simulink model "Simulink_mg_1234_with_DistributedControl_ControlConmutado"  (R2018a)
settings: Solver=VariableStepAuto  StartTime=0.0  StopTime=50  FixedStep=1e-6  MaxStep=1e-3  RelTol=1e-3
values from neighbouring files (symbols this model uses):
  aij = 1    [Simulation_Base_4_mg.m]    (also in Simulation_alpha_vs_tau.m)
  aij_1 = 10    [Simulation_Base_4_mg.m]    (also in Simulation_alpha_vs_tau.m)
  aij_2 = 10    [Simulation_Base_4_mg.m]    (also in Simulation_alpha_vs_tau.m)
  aij_3 = 10    [Simulation_Base_4_mg.m]    (also in Simulation_alpha_vs_tau.m)
  aij_4 = 10    [Simulation_Base_4_mg.m]    (also in Simulation_alpha_vs_tau.m)
  C_mg_1 = Ctot .* dist    [Simulation_Base_4_mg.m]    (also in Simulation_alpha_vs_tau.m)
  C_mg_2 = Ctot .* dist    [Simulation_Base_4_mg.m]    (also in Simulation_alpha_vs_tau.m)
  C_mg_3 = Ctot .* dist    [Simulation_Base_4_mg.m]    (also in Simulation_alpha_vs_tau.m)
  C_mg_4 = Ctot .* dist    [Simulation_Base_4_mg.m]    (also in Simulation_alpha_vs_tau.m)
  g12 = 1.2    [Simulation_Base_4_mg.m]    (also in Simulation_alpha_vs_tau.m)
  g12_1 = 1/r_jk    (= 10)    [Simulation_Base_4_mg.m]    (also in Simulation_alpha_vs_tau.m)
  g12_2 = 1/r_jk    (= 10)    [Simulation_Base_4_mg.m]    (also in Simulation_alpha_vs_tau.m)
  g12_3 = 1/r_jk    (= 10)    [Simulation_Base_4_mg.m]    (also in Simulation_alpha_vs_tau.m)
  g12_4 = 1/r_jk    (= 10)    [Simulation_Base_4_mg.m]    (also in Simulation_alpha_vs_tau.m)
  g13 = ((0.383+1.756) / (0.383*1.756))^(-1)    (= 0.31442169238)    [Simulation_Base_4_mg.m]    (also in Simulation_alpha_vs_tau.m)
  g13_1 = 1/r_jk    (= 10)    [Simulation_Base_4_mg.m]    (also in Simulation_alpha_vs_tau.m)
  g13_3 = 1/r_jk    (= 10)    [Simulation_Base_4_mg.m]    (also in Simulation_alpha_vs_tau.m)
  g13_4 = 1/r_jk    (= 10)    [Simulation_Base_4_mg.m]    (also in Simulation_alpha_vs_tau.m)
  g23_1 = 1/r_jk    (= 10)    [Simulation_Base_4_mg.m]    (also in Simulation_alpha_vs_tau.m)
  g23_4 = 1/r_jk    (= 10)    [Simulation_Base_4_mg.m]    (also in Simulation_alpha_vs_tau.m)
  g24 = 1.55    [Simulation_Base_4_mg.m]    (also in Simulation_alpha_vs_tau.m)
  g24_3 = 1/r_jk    (= 10)    [Simulation_Base_4_mg.m]    (also in Simulation_alpha_vs_tau.m)
  g24_4 = 1/r_jk    (= 10)    [Simulation_Base_4_mg.m]    (also in Simulation_alpha_vs_tau.m)
  g34 = 0.75    [Simulation_Base_4_mg.m]    (also in Simulation_alpha_vs_tau.m)
  g34_3 = 1/r_jk    (= 10)    [Simulation_Base_4_mg.m]    (also in Simulation_alpha_vs_tau.m)
  g34_4 = 1/r_jk    (= 10)    [Simulation_Base_4_mg.m]    (also in Simulation_alpha_vs_tau.m)
  h = 0.99    [Simulation_Base_4_mg.m]    (also in Simulation_alpha_vs_tau.m)
  I_rate = [100,50,33,33]    [Simulation_Base_4_mg.m]    (also in Simulation_alpha_vs_tau.m)
  I_rate_1 = [5, 2.5, 2.5]    [Simulation_Base_4_mg.m]    (also in Simulation_alpha_vs_tau.m)
  I_rate_2 = [2.5, 5]    [Simulation_Base_4_mg.m]    (also in Simulation_alpha_vs_tau.m)
  I_rate_3 = [4, 3, 2, 1]    [Simulation_Base_4_mg.m]    (also in Simulation_alpha_vs_tau.m)
  I_rate_4 = [4, 3, 2, 1]    [Simulation_Base_4_mg.m]    (also in Simulation_alpha_vs_tau.m)
  k_ii = 60    [Simulation_Base_4_mg.m]    (also in Simulation_alpha_vs_tau.m)
  k_ii2 = 10    [Simulation_Base_4_mg.m]    (also in Simulation_alpha_vs_tau.m)
  k_ii_1 = 1000    [Simulation_Base_4_mg.m]    (also in Simulation_alpha_vs_tau.m)
  k_ii_2 = 1000    [Simulation_Base_4_mg.m]    (also in Simulation_alpha_vs_tau.m)
  k_ii_3 = 1000    [Simulation_Base_4_mg.m]    (also in Simulation_alpha_vs_tau.m)
  k_ii_4 = 1000    [Simulation_Base_4_mg.m]    (also in Simulation_alpha_vs_tau.m)
  k_iv = 3    [Simulation_Base_4_mg.m]    (also in Simulation_alpha_vs_tau.m = 1)
  k_iv_1 = 30    [Simulation_Base_4_mg.m]    (also in Simulation_alpha_vs_tau.m)
  k_iv_2 = 30    [Simulation_Base_4_mg.m]    (also in Simulation_alpha_vs_tau.m)
  k_iv_3 = 30    [Simulation_Base_4_mg.m]    (also in Simulation_alpha_vs_tau.m)
  k_iv_4 = 30    [Simulation_Base_4_mg.m]    (also in Simulation_alpha_vs_tau.m)
  k_pi = 30    [Simulation_Base_4_mg.m]    (also in Simulation_alpha_vs_tau.m = 25)
  k_pi2 = 0.5    [Simulation_Base_4_mg.m]    (also in Simulation_alpha_vs_tau.m)
  k_pi_1 = 10    [Simulation_Base_4_mg.m]    (also in Simulation_alpha_vs_tau.m)
  k_pi_2 = 10    [Simulation_Base_4_mg.m]    (also in Simulation_alpha_vs_tau.m)
  k_pi_3 = 10    [Simulation_Base_4_mg.m]    (also in Simulation_alpha_vs_tau.m)
  k_pi_4 = 10    [Simulation_Base_4_mg.m]    (also in Simulation_alpha_vs_tau.m)
  kd_1 = [5, 2.5, 2.5]    [Simulation_Base_4_mg.m]    (also in Simulation_alpha_vs_tau.m)
  kd_2 = [2.5, 50]    [Simulation_Base_4_mg.m]    (also in Simulation_alpha_vs_tau.m)
  kd_3 = [4, 3, 2, 1]    [Simulation_Base_4_mg.m]    (also in Simulation_alpha_vs_tau.m)
  kd_4 = [4, 3, 2, 1]    [Simulation_Base_4_mg.m]    (also in Simulation_alpha_vs_tau.m)
  L_mg_1 = ones(n) .* n .* Ltot    [Simulation_Base_4_mg.m]    (also in Simulation_alpha_vs_tau.m)
  L_mg_2 = ones(n) .* n .* Ltot    [Simulation_Base_4_mg.m]    (also in Simulation_alpha_vs_tau.m)
  L_mg_3 = ones(n) .* n .* Ltot    [Simulation_Base_4_mg.m]    (also in Simulation_alpha_vs_tau.m)
  L_mg_4 = ones(n) .* n .* Ltot    [Simulation_Base_4_mg.m]    (also in Simulation_alpha_vs_tau.m)
  P_load_vertex_1 = [   P_load_vertex_1;                                                 P_aux(i1,1) , P_aux(i2,2) , P_aux(i3,3) ]    [Simulation_Base_4_mg.m]    (also in Simulation_alpha_vs_tau.m)
  P_load_vertex_2 = [   P_load_vertex_2;                                                 P_aux(i1,1) , P_aux(i2,2) ]    [Simulation_Base_4_mg.m]    (also in Simulation_alpha_vs_tau.m)
  P_load_vertex_3 = [   P_load_vertex_3;                                                 P_aux(i1,1) , P_aux(i2,2) , P_aux(i3,3), P_aux(i4,4) ]    [Simulation_Base_4_mg.m]    (also in Simulation_alpha_vs_tau.m)
  P_load_vertex_4 = [   P_load_vertex_4;                                                 P_aux(i1,1) , P_aux(i2,2) , P_aux(i3,3), P_aux(i4,4) ]    [Simulation_Base_4_mg.m]    (also in Simulation_alpha_vs_tau.m)
  r_d0 = 1.3    [Simulation_Base_4_mg.m]    (also in Simulation_alpha_vs_tau.m)
  rd_mg_1 = n^2 * rtot .* dist    [Simulation_Base_4_mg.m]    (also in Simulation_alpha_vs_tau.m)
  rd_mg_2 = n^2 * rtot .* dist    [Simulation_Base_4_mg.m]    (also in Simulation_alpha_vs_tau.m)
  rd_mg_3 = n^2 * rtot .* dist    [Simulation_Base_4_mg.m]    (also in Simulation_alpha_vs_tau.m)
  rd_mg_4 = n^2 * rtot .* dist    [Simulation_Base_4_mg.m]    (also in Simulation_alpha_vs_tau.m)
  tau = 0.5    [Simulation_Base_4_mg.m]    (also in Simulation_alpha_vs_tau.m = 0.066)
  time_1 = 0.5    [Simulation_Base_4_mg.m]    (also in Simulation_alpha_vs_tau.m)
  time_2 = 15    [Simulation_Base_4_mg.m]    (also in Simulation_alpha_vs_tau.m = 5)
  time_4 = 5    [Simulation_Base_4_mg.m]    (also in Simulation_alpha_vs_tau.m = 15)
  time_6 = 50    [Simulation_Base_4_mg.m]    (also in Simulation_alpha_vs_tau.m = 13)
  time_7 = 50    [Simulation_Base_4_mg.m]    (also in Simulation_alpha_vs_tau.m = 100)
  time_8 = 50    [Simulation_Base_4_mg.m]    (also in Simulation_alpha_vs_tau.m = 100)
  time_9 = 100    [Simulation_Base_4_mg.m]    (also in Simulation_alpha_vs_tau.m)
  time_a_down = 100    [Simulation_alpha_vs_tau.m]
  time_a_up = 100    [Simulation_alpha_vs_tau.m]
  time_tau_down = 25    [Simulation_alpha_vs_tau.m]
  V_ref = 1050    [Simulation_Base_4_mg.m]    (also in Simulation_alpha_vs_tau.m)
undefined symbols (not defined in the file or in its folder): Zout_den_source, Zout_num_source
libraries: fl_lib x128, nesl_utility x89, elec_lib x26
(part 1 of 2)
settings Model: Creator=carna  LastModifiedBy=carna
settings SolverCC: ZeroCrossAlgorithm=Adaptive

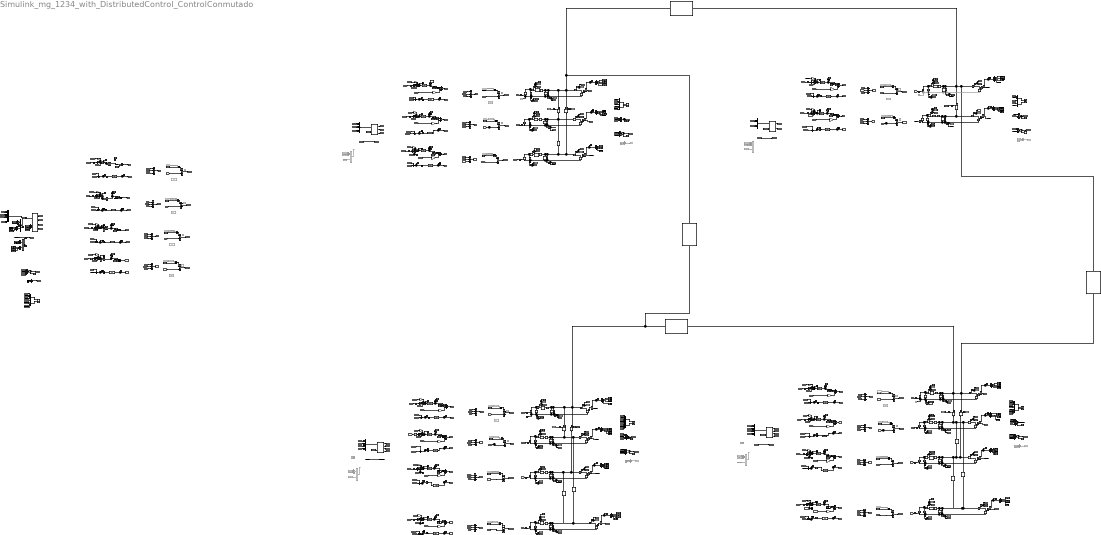
== system Simulink_mg_1234_with_DistributedControl_ControlConmutado ==
  note: Delta v 1
  note: Delta v 2
  note: DELTA I
  note: Delta R droop
  note: DELTA I
  note: Delta R droop
  note: Delta R droop
  note: DELTA I
  note: V MG
  note: I MG
  note: DELTA I
  note: Delta v 3
  note: Delta R droop
  note: Delta v 1
  note: Delta v 2
  note: DELTA I
  note: Delta R droop
  note: DELTA I
  note: Delta R droop
  note: Delta R droop
  note: DELTA I
  note: V MG
  note: I MG
  note: DELTA I
  note: Delta v 3
  note: Delta R droop
  note: Delta v 1
  note: Delta v 2
  note: DELTA I
  note: Delta R droop
  note: DELTA I
  note: Delta R droop
  note: Delta R droop
  note: DELTA I
  note: V MG
  note: I MG
  note: Delta v 1
  note: Delta v 2
  note: Delta R droop
  note: DELTA I
  note: Delta R droop
  note: DELTA I
  note: V MG
  note: I MG
  note: Delta v 1
  note: Delta R droop
  note: DELTA I
  note: V MG
  note: Delta v 1
  note: Delta R droop
  note: DELTA I
  note: Delta v 1
  note: Delta R droop
  note: DELTA I
  note: Delta v 1
  note: Delta R droop
  note: DELTA I
  Add{1,8,24,32,46..47,54,69} (8 alike) : Sum  Commented=on
  Add{2..4,9..13,15..16,19..20,36..38,61..62,73} (18 alike) : Sum  Inputs=++++
  Add{5,14,17,25..26,31,33,40..41,49,55,60,64..65,70,76,78} (17 alike) : Sum  Inputs=-+
  Add{6,18,22,27,29,39,43..44,50,52,57,63,67,71,75,77,79} (17 alike) : Sum  Inputs=-++
  Add{7,21,23,28,30,42,45,48,51,53,56,58..59,66,68,72,74,80} (18 alike) : Sum
  Add{34..35,81..83} (5 alike) : Sum  Inputs=+++
  C bus 1 : elec_lib/Passive Devices/Capacitor  enable_table=0  c=C_mg_3(1) F  Cvec=[1.0e-5, 1.0e-6] F  Vvec=[0.0, 10.0] V  CV_table_symmetry=1  C_tol=5  enable_C_tol=0  tol_distribution=1  nSigma=4  r=1e-6 Ohm  g=0 1/Ohm  enable_operating_limits=0  operating_limit_action=2  max_working_voltage_range=[-25.0, 25.0] V  power_rating=1 W  enable_faults=0  fault_action=1  Cscale_faulted=100  R_faulted=1e-3 Ohm  G_faulted=0 1/Ohm  tau_fault=1e-3 s  enable_temporal_fault=0  t_fault=1 s  enable_behavioral_fault=0  max_permissible_voltage_range=[-100.0, 100.0] V  t_fail_on_voltage=1 s  i_specify=off  i_priority=None  i=0 A  i_nominal_specify=off  i_nominal_unit=A  i_nominal_value=1  v_specify=off  v_priority=None  v=0 V  v_nominal_specify=off  v_nominal_unit=V  v_nominal_value=1  vc_specify=off  vc_priority=High  vc=0 V  vc_nominal_specify=off  vc_nominal_unit=V  vc_nominal_value=1
  C bus 10 : elec_lib/Passive Devices/Capacitor  enable_table=0  c=C_mg_1(2) F  Cvec=[1.0e-5, 1.0e-6] F  Vvec=[0.0, 10.0] V  CV_table_symmetry=1  C_tol=5  enable_C_tol=0  tol_distribution=1  nSigma=4  r=1e-6 Ohm  g=0 1/Ohm  enable_operating_limits=0  operating_limit_action=2  max_working_voltage_range=[-25.0, 25.0] V  power_rating=1 W  enable_faults=0  fault_action=1  Cscale_faulted=100  R_faulted=1e-3 Ohm  G_faulted=0 1/Ohm  tau_fault=1e-3 s  enable_temporal_fault=0  t_fault=1 s  enable_behavioral_fault=0  max_permissible_voltage_range=[-100.0, 100.0] V  t_fail_on_voltage=1 s  i_specify=off  i_priority=None  i=0 A  i_nominal_specify=off  i_nominal_unit=A  i_nominal_value=1  v_specify=on  v_priority=None  v=990 V  v_nominal_specify=off  v_nominal_unit=V  v_nominal_value=1  vc_specify=off  vc_priority=High  vc=0 V  vc_nominal_specify=off  vc_nominal_unit=V  vc_nominal_value=1
  C bus 11 : elec_lib/Passive Devices/Capacitor  enable_table=0  c=C_mg_1(3) F  Cvec=[1.0e-5, 1.0e-6] F  Vvec=[0.0, 10.0] V  CV_table_symmetry=1  C_tol=5  enable_C_tol=0  tol_distribution=1  nSigma=4  r=1e-6 Ohm  g=0 1/Ohm  enable_operating_limits=0  operating_limit_action=2  max_working_voltage_range=[-25.0, 25.0] V  power_rating=1 W  enable_faults=0  fault_action=1  Cscale_faulted=100  R_faulted=1e-3 Ohm  G_faulted=0 1/Ohm  tau_fault=1e-3 s  enable_temporal_fault=0  t_fault=1 s  enable_behavioral_fault=0  max_permissible_voltage_range=[-100.0, 100.0] V  t_fail_on_voltage=1 s  i_specify=off  i_priority=None  i=0 A  i_nominal_specify=off  i_nominal_unit=A  i_nominal_value=1  v_specify=on  v_priority=None  v=990 V  v_nominal_specify=off  v_nominal_unit=V  v_nominal_value=1  vc_specify=off  vc_priority=High  vc=0 V  vc_nominal_specify=off  vc_nominal_unit=V  vc_nominal_value=1
  C bus 12 : elec_lib/Passive Devices/Capacitor  enable_table=0  c=C_mg_2(2) F  Cvec=[1.0e-5, 1.0e-6] F  Vvec=[0.0, 10.0] V  CV_table_symmetry=1  C_tol=5  enable_C_tol=0  tol_distribution=1  nSigma=4  r=1e-6 Ohm  g=0 1/Ohm  enable_operating_limits=0  operating_limit_action=2  max_working_voltage_range=[-25.0, 25.0] V  power_rating=1 W  enable_faults=0  fault_action=1  Cscale_faulted=100  R_faulted=1e-3 Ohm  G_faulted=0 1/Ohm  tau_fault=1e-3 s  enable_temporal_fault=0  t_fault=1 s  enable_behavioral_fault=0  max_permissible_voltage_range=[-100.0, 100.0] V  t_fail_on_voltage=1 s  i_specify=off  i_priority=None  i=0 A  i_nominal_specify=off  i_nominal_unit=A  i_nominal_value=1  v_specify=on  v_priority=None  v=990 V  v_nominal_specify=off  v_nominal_unit=V  v_nominal_value=1  vc_specify=off  vc_priority=High  vc=0 V  vc_nominal_specify=off  vc_nominal_unit=V  vc_nominal_value=1
  C bus 14 : elec_lib/Passive Devices/Capacitor  enable_table=0  c=C_mg_2(1) F  Cvec=[1.0e-5, 1.0e-6] F  Vvec=[0.0, 10.0] V  CV_table_symmetry=1  C_tol=5  enable_C_tol=0  tol_distribution=1  nSigma=4  r=1e-6 Ohm  g=0 1/Ohm  enable_operating_limits=0  operating_limit_action=2  max_working_voltage_range=[-25.0, 25.0] V  power_rating=1 W  enable_faults=0  fault_action=1  Cscale_faulted=100  R_faulted=1e-3 Ohm  G_faulted=0 1/Ohm  tau_fault=1e-3 s  enable_temporal_fault=0  t_fault=1 s  enable_behavioral_fault=0  max_permissible_voltage_range=[-100.0, 100.0] V  t_fail_on_voltage=1 s  i_specify=off  i_priority=None  i=0 A  i_nominal_specify=off  i_nominal_unit=A  i_nominal_value=1  v_specify=on  v_priority=None  v=990 V  v_nominal_specify=off  v_nominal_unit=V  v_nominal_value=1  vc_specify=off  vc_priority=High  vc=0 V  vc_nominal_specify=off  vc_nominal_unit=V  vc_nominal_value=1
  C bus 2 : elec_lib/Passive Devices/Capacitor  enable_table=0  c=C_mg_3(2) F  Cvec=[1.0e-5, 1.0e-6] F  Vvec=[0.0, 10.0] V  CV_table_symmetry=1  C_tol=5  enable_C_tol=0  tol_distribution=1  nSigma=4  r=1e-6 Ohm  g=0 1/Ohm  enable_operating_limits=0  operating_limit_action=2  max_working_voltage_range=[-25.0, 25.0] V  power_rating=1 W  enable_faults=0  fault_action=1  Cscale_faulted=100  R_faulted=1e-3 Ohm  G_faulted=0 1/Ohm  tau_fault=1e-3 s  enable_temporal_fault=0  t_fault=1 s  enable_behavioral_fault=0  max_permissible_voltage_range=[-100.0, 100.0] V  t_fail_on_voltage=1 s  i_specify=off  i_priority=None  i=0 A  i_nominal_specify=off  i_nominal_unit=A  i_nominal_value=1  v_specify=off  v_priority=None  v=0 V  v_nominal_specify=off  v_nominal_unit=V  v_nominal_value=1  vc_specify=off  vc_priority=High  vc=0 V  vc_nominal_specify=off  vc_nominal_unit=V  vc_nominal_value=1
  C bus 3 : elec_lib/Passive Devices/Capacitor  enable_table=0  c=C_mg_3(3) F  Cvec=[1.0e-5, 1.0e-6] F  Vvec=[0.0, 10.0] V  CV_table_symmetry=1  C_tol=5  enable_C_tol=0  tol_distribution=1  nSigma=4  r=1e-6 Ohm  g=0 1/Ohm  enable_operating_limits=0  operating_limit_action=2  max_working_voltage_range=[-25.0, 25.0] V  power_rating=1 W  enable_faults=0  fault_action=1  Cscale_faulted=100  R_faulted=1e-3 Ohm  G_faulted=0 1/Ohm  tau_fault=1e-3 s  enable_temporal_fault=0  t_fault=1 s  enable_behavioral_fault=0  max_permissible_voltage_range=[-100.0, 100.0] V  t_fail_on_voltage=1 s  i_specify=off  i_priority=None  i=0 A  i_nominal_specify=off  i_nominal_unit=A  i_nominal_value=1  v_specify=off  v_priority=None  v=0 V  v_nominal_specify=off  v_nominal_unit=V  v_nominal_value=1  vc_specify=off  vc_priority=High  vc=0 V  vc_nominal_specify=off  vc_nominal_unit=V  vc_nominal_value=1
  C bus 4 : elec_lib/Passive Devices/Capacitor  enable_table=0  c=C_mg_3(4) F  Cvec=[1.0e-5, 1.0e-6] F  Vvec=[0.0, 10.0] V  CV_table_symmetry=1  C_tol=5  enable_C_tol=0  tol_distribution=1  nSigma=4  r=1e-6 Ohm  g=0 1/Ohm  enable_operating_limits=0  operating_limit_action=2  max_working_voltage_range=[-25.0, 25.0] V  power_rating=1 W  enable_faults=0  fault_action=1  Cscale_faulted=100  R_faulted=1e-3 Ohm  G_faulted=0 1/Ohm  tau_fault=1e-3 s  enable_temporal_fault=0  t_fault=1 s  enable_behavioral_fault=0  max_permissible_voltage_range=[-100.0, 100.0] V  t_fail_on_voltage=1 s  i_specify=off  i_priority=None  i=0 A  i_nominal_specify=off  i_nominal_unit=A  i_nominal_value=1  v_specify=off  v_priority=None  v=0 V  v_nominal_specify=off  v_nominal_unit=V  v_nominal_value=1  vc_specify=off  vc_priority=High  vc=0 V  vc_nominal_specify=off  vc_nominal_unit=V  vc_nominal_value=1
  C bus 5 : elec_lib/Passive Devices/Capacitor  enable_table=0  c=C_mg_3(1) F  Cvec=[1.0e-5, 1.0e-6] F  Vvec=[0.0, 10.0] V  CV_table_symmetry=1  C_tol=5  enable_C_tol=0  tol_distribution=1  nSigma=4  r=1e-6 Ohm  g=0 1/Ohm  enable_operating_limits=0  operating_limit_action=2  max_working_voltage_range=[-25.0, 25.0] V  power_rating=1 W  enable_faults=0  fault_action=1  Cscale_faulted=100  R_faulted=1e-3 Ohm  G_faulted=0 1/Ohm  tau_fault=1e-3 s  enable_temporal_fault=0  t_fault=1 s  enable_behavioral_fault=0  max_permissible_voltage_range=[-100.0, 100.0] V  t_fail_on_voltage=1 s  i_specify=off  i_priority=None  i=0 A  i_nominal_specify=off  i_nominal_unit=A  i_nominal_value=1  v_specify=off  v_priority=None  v=0 V  v_nominal_specify=off  v_nominal_unit=V  v_nominal_value=1  vc_specify=off  vc_priority=High  vc=0 V  vc_nominal_specify=off  vc_nominal_unit=V  vc_nominal_value=1
  C bus 6 : elec_lib/Passive Devices/Capacitor  enable_table=0  c=C_mg_4(2) F  Cvec=[1.0e-5, 1.0e-6] F  Vvec=[0.0, 10.0] V  CV_table_symmetry=1  C_tol=5  enable_C_tol=0  tol_distribution=1  nSigma=4  r=1e-6 Ohm  g=0 1/Ohm  enable_operating_limits=0  operating_limit_action=2  max_working_voltage_range=[-25.0, 25.0] V  power_rating=1 W  enable_faults=0  fault_action=1  Cscale_faulted=100  R_faulted=1e-3 Ohm  G_faulted=0 1/Ohm  tau_fault=1e-3 s  enable_temporal_fault=0  t_fault=1 s  enable_behavioral_fault=0  max_permissible_voltage_range=[-100.0, 100.0] V  t_fail_on_voltage=1 s  i_specify=off  i_priority=None  i=0 A  i_nominal_specify=off  i_nominal_unit=A  i_nominal_value=1  v_specify=off  v_priority=None  v=0 V  v_nominal_specify=off  v_nominal_unit=V  v_nominal_value=1  vc_specify=off  vc_priority=High  vc=0 V  vc_nominal_specify=off  vc_nominal_unit=V  vc_nominal_value=1
  C bus 7 : elec_lib/Passive Devices/Capacitor  enable_table=0  c=C_mg_3(3) F  Cvec=[1.0e-5, 1.0e-6] F  Vvec=[0.0, 10.0] V  CV_table_symmetry=1  C_tol=5  enable_C_tol=0  tol_distribution=1  nSigma=4  r=1e-6 Ohm  g=0 1/Ohm  enable_operating_limits=0  operating_limit_action=2  max_working_voltage_range=[-25.0, 25.0] V  power_rating=1 W  enable_faults=0  fault_action=1  Cscale_faulted=100  R_faulted=1e-3 Ohm  G_faulted=0 1/Ohm  tau_fault=1e-3 s  enable_temporal_fault=0  t_fault=1 s  enable_behavioral_fault=0  max_permissible_voltage_range=[-100.0, 100.0] V  t_fail_on_voltage=1 s  i_specify=off  i_priority=None  i=0 A  i_nominal_specify=off  i_nominal_unit=A  i_nominal_value=1  v_specify=off  v_priority=None  v=0 V  v_nominal_specify=off  v_nominal_unit=V  v_nominal_value=1  vc_specify=off  vc_priority=High  vc=0 V  vc_nominal_specify=off  vc_nominal_unit=V  vc_nominal_value=1
  C bus 8 : elec_lib/Passive Devices/Capacitor  enable_table=0  c=C_mg_4(4) F  Cvec=[1.0e-5, 1.0e-6] F  Vvec=[0.0, 10.0] V  CV_table_symmetry=1  C_tol=5  enable_C_tol=0  tol_distribution=1  nSigma=4  r=1e-6 Ohm  g=0 1/Ohm  enable_operating_limits=0  operating_limit_action=2  max_working_voltage_range=[-25.0, 25.0] V  power_rating=1 W  enable_faults=0  fault_action=1  Cscale_faulted=100  R_faulted=1e-3 Ohm  G_faulted=0 1/Ohm  tau_fault=1e-3 s  enable_temporal_fault=0  t_fault=1 s  enable_behavioral_fault=0  max_permissible_voltage_range=[-100.0, 100.0] V  t_fail_on_voltage=1 s  i_specify=off  i_priority=None  i=0 A  i_nominal_specify=off  i_nominal_unit=A  i_nominal_value=1  v_specify=off  v_priority=None  v=0 V  v_nominal_specify=off  v_nominal_unit=V  v_nominal_value=1  vc_specify=off  vc_priority=High  vc=0 V  vc_nominal_specify=off  vc_nominal_unit=V  vc_nominal_value=1
  C bus 9 : elec_lib/Passive Devices/Capacitor  enable_table=0  c=C_mg_1(1) F  Cvec=[1.0e-5, 1.0e-6] F  Vvec=[0.0, 10.0] V  CV_table_symmetry=1  C_tol=5  enable_C_tol=0  tol_distribution=1  nSigma=4  r=1e-6 Ohm  g=0 1/Ohm  enable_operating_limits=0  operating_limit_action=2  max_working_voltage_range=[-25.0, 25.0] V  power_rating=1 W  enable_faults=0  fault_action=1  Cscale_faulted=100  R_faulted=1e-3 Ohm  G_faulted=0 1/Ohm  tau_fault=1e-3 s  enable_temporal_fault=0  t_fault=1 s  enable_behavioral_fault=0  max_permissible_voltage_range=[-100.0, 100.0] V  t_fail_on_voltage=1 s  i_specify=off  i_priority=None  i=0 A  i_nominal_specify=off  i_nominal_unit=A  i_nominal_value=1  v_specify=on  v_priority=None  v=990 V  v_nominal_specify=off  v_nominal_unit=V  v_nominal_value=1  vc_specify=off  vc_priority=High  vc=0 V  vc_nominal_specify=off  vc_nominal_unit=V  vc_nominal_value=1
  Close loop equivalent{1..4} (4 alike) : TransferFcn  Numerator=[0 k_iv_3 ]  Denominator=[1 0]
  Close loop equivalent{6,9..11,14,18,20..23,25,29..31,35,38,41} (17 alike) : TransferFcn  Commented=on  Numerator=Zout_num_source  Denominator=Zout_den_source
  Close loop equivalent{5,8,12..13} (4 alike) : TransferFcn  Numerator=[0 k_iv_4 ]  Denominator=[1 0]
  Close loop equivalent15 : TransferFcn  Numerator=[0 k_iv_1 ]  Denominator=[1 0]
  Close loop equivalent{7,16,19,26..27,34,37,40} (8 alike) : TransferFcn  Commented=on  Numerator=[1 ]  Denominator=[tau 1]
  Close loop equivalent17 : TransferFcn  Numerator=[0 k_iv_1 ]  Denominator=[1 0]
  Close loop equivalent24 : TransferFcn  Numerator=[0 k_iv_1 ]  Denominator=[1 0]
  Close loop equivalent28 : TransferFcn  Numerator=[0 k_iv_2 ]  Denominator=[1 0]
  Close loop equivalent32 : TransferFcn  Numerator=[0 k_iv_2 ]  Denominator=[1 0]
  Close loop equivalent{33,36,39,42} (4 alike) : TransferFcn  Numerator=[0 k_iv ]  Denominator=[1 0]
  Constant{1,6,23,27} (4 alike) : Constant  Commented=on  Value=tau/2
  Constant{2..3,7..16,19..22,24..26,28..31,34..38,44..49} (34 alike) : Constant  Value=0
  Constant{4,17,32,39} (4 alike) : Constant  Commented=on  Value=V_ref
  Constant18 : Constant  Value=aij_4
  Constant33 : Constant  Value=aij_1
  Constant40 : Constant  Value=aij_2
  Constant41 : Constant  Value=tau*3/4
  Constant42 : Constant  Value=aij
  Constant43 : Constant  Value=V_ref
  Constant5 : Constant  Value=aij_3
  Constant50 : Constant  Value=tau*3/4
  Controlled Current Source{1..13} (13 alike) : fl_lib/Electrical/Electrical Sources/Controlled Current Source
  Controlled Voltage Source{,1..12} (13 alike) : fl_lib/Electrical/Electrical Sources/Controlled Voltage Source
  Current cloop transfer- Transport Delay{1..12} (12 alike) : TransportDelay  Commented=on  DelayTime=0.1e-3
  Current load {1..12,14} (13 alike) : fl_lib/Electrical/Electrical Sensors/Current Sensor
  Current output {1..19,21} (20 alike) : fl_lib/Electrical/Electrical Sensors/Current Sensor
  Derivative : Derivative  Commented=on
  Derivative1 : Derivative  Commented=on
  Display{,1..41,43..47,49..53,55..57,59,61..63} (59 alike) : Display
  Divide{1..13} (13 alike) : Product  Inputs=*/
  Electrical Reference{,1..10,12..13} (13 alike) : fl_lib/Electrical/Electrical Elements/Electrical Reference
  From{47,104,144,172} (4 alike) : From  Commented=on  GotoTag=io_source_2
  From{54,113,151,161,182,247,256,265} (8 alike) : From  Commented=on  GotoTag=io_source_1
  From{18,56,77,116,153} (5 alike) : From  Commented=on  GotoTag=io_source_3
  Gain1 : Gain  Gain=1/I_rate_3(4)
  Gain10 : Gain  Gain=r_d0/kd_4(1)
  Gain11 : Gain  Gain=r_d0/kd_4(4)
  Gain12 : Gain  Gain=1/I_rate_3(2)
  Gain13 : Gain  Gain=1/I_rate_3(3)
  Gain14 : Gain  Gain=1/4
  Gain15 : Gain  Gain=r_d0/kd_3(2)
  Gain16 : Gain  Gain=r_d0/kd_3(3)
  Gain17 : Gain  Gain=1/I_rate_3(1)
  Gain18 : Gain  Gain=r_d0/kd_3(1)
  Gain19 : Gain  Gain=1/I_rate_2(2)
  Gain2 : Gain  Gain=r_d0/kd_3(4)
  Gain20 : Gain  Gain=1/I_rate_1(2)
  Gain21 : Gain  Gain=1/I_rate_1(3)
  Gain22 : Gain  Gain=r_d0/kd_1(2)
  Gain23 : Gain  Gain=r_d0/kd_1(3)
  Gain24 : Gain  Gain=1/I_rate_1(1)
  Gain25 : Gain  Gain=r_d0/kd_1(1)
  Gain26 : Gain  Gain=1/I_rate(1)
  Gain27 : Gain  Gain=1/3
  Gain28 : Gain  Gain=r_d0/kd_2(2)
  Gain29 : Gain  Gain=1/I_rate(2)
  Gain3 : Gain  Gain=1/I_rate_4(4)
  Gain30 : Gain  Gain=1/I_rate_2(1)
  Gain31 : Gain  Gain=r_d0/kd_2(1)
  Gain32 : Gain  Gain=1/2
  Gain33 : Gain  Gain=1/4
  Gain34 : Gain  Gain=1/I_rate(3)
  Gain35 : Gain  Gain=1/I_rate(4)
  Gain4 : Gain  Gain=1/I_rate_4(2)
  Gain5 : Gain  Gain=1/4
  Gain6 : Gain  Gain=1/I_rate_4(3)
  Gain7 : Gain  Gain=r_d0/kd_4(2)
  Gain8 : Gain  Gain=r_d0/kd_4(3)
  Gain9 : Gain  Gain=1/I_rate_4(1)
  Goto{29,44,94,106} (4 alike) : Goto  Commented=on  GotoTag=V_REF_c
  Integrator{1..17} (17 alike) : Integrator
  L serie 1 : elec_lib/Passive Devices/Inductor  l=L_mg_3(1) H  L_tol=20  enable_L_tol=0  tol_distribution=1  nSigma=4  r=0 Ohm  g=1e-9 1/Ohm  enable_operating_limits=0  operating_limit_action=2  max_working_current=1 A  power_rating=1 W  enable_faults=0  fault_action=1  lambdaPercent=50  k_faulted=0.9999  turnsShort=0  openCct=0  groundShort=0  groundShortG=0 1/Ohm  tau_fault=1e-3 s  enable_temporal_fault=0  t_fault=1 s  enable_behavioral_fault=0  max_permissible_voltage=100 V  n_fail_on_voltage=1  max_permissible_current=1 A  t_fail_on_current=1 s  i_L_specify=off  i_L_priority=High  i_L=0 A  i_L_nominal_specify=off  i_L_nominal_unit=A  i_L_nominal_value=1
      settings: SourceProductName=Simscape Electronics  SourceProductBaseCode=SN
  L serie 10 : elec_lib/Passive Devices/Inductor  l=L_mg_1(2) H  L_tol=20  enable_L_tol=0  tol_distribution=1  nSigma=4  r=0 Ohm  g=1e-9 1/Ohm  enable_operating_limits=0  operating_limit_action=2  max_working_current=1 A  power_rating=1 W  enable_faults=0  fault_action=1  lambdaPercent=50  k_faulted=0.9999  turnsShort=0  openCct=0  groundShort=0  groundShortG=0 1/Ohm  tau_fault=1e-3 s  enable_temporal_fault=0  t_fault=1 s  enable_behavioral_fault=0  max_permissible_voltage=100 V  n_fail_on_voltage=1  max_permissible_current=1 A  t_fail_on_current=1 s  i_L_specify=off  i_L_priority=High  i_L=0 A  i_L_nominal_specify=off  i_L_nominal_unit=A  i_L_nominal_value=1
      settings: SourceProductName=Simscape Electronics  SourceProductBaseCode=SN
  L serie 11 : elec_lib/Passive Devices/Inductor  l=L_mg_1(3) H  L_tol=20  enable_L_tol=0  tol_distribution=1  nSigma=4  r=0 Ohm  g=1e-9 1/Ohm  enable_operating_limits=0  operating_limit_action=2  max_working_current=1 A  power_rating=1 W  enable_faults=0  fault_action=1  lambdaPercent=50  k_faulted=0.9999  turnsShort=0  openCct=0  groundShort=0  groundShortG=0 1/Ohm  tau_fault=1e-3 s  enable_temporal_fault=0  t_fault=1 s  enable_behavioral_fault=0  max_permissible_voltage=100 V  n_fail_on_voltage=1  max_permissible_current=1 A  t_fail_on_current=1 s  i_L_specify=off  i_L_priority=High  i_L=0 A  i_L_nominal_specify=off  i_L_nominal_unit=A  i_L_nominal_value=1
      settings: SourceProductName=Simscape Electronics  SourceProductBaseCode=SN
  L serie 12 : elec_lib/Passive Devices/Inductor  l=L_mg_2(2) H  L_tol=20  enable_L_tol=0  tol_distribution=1  nSigma=4  r=0 Ohm  g=1e-9 1/Ohm  enable_operating_limits=0  operating_limit_action=2  max_working_current=1 A  power_rating=1 W  enable_faults=0  fault_action=1  lambdaPercent=50  k_faulted=0.9999  turnsShort=0  openCct=0  groundShort=0  groundShortG=0 1/Ohm  tau_fault=1e-3 s  enable_temporal_fault=0  t_fault=1 s  enable_behavioral_fault=0  max_permissible_voltage=100 V  n_fail_on_voltage=1  max_permissible_current=1 A  t_fail_on_current=1 s  i_L_specify=off  i_L_priority=High  i_L=0 A  i_L_nominal_specify=off  i_L_nominal_unit=A  i_L_nominal_value=1
      settings: SourceProductName=Simscape Electronics  SourceProductBaseCode=SN
  L serie 14 : elec_lib/Passive Devices/Inductor  l=L_mg_2(1) H  L_tol=20  enable_L_tol=0  tol_distribution=1  nSigma=4  r=0 Ohm  g=1e-9 1/Ohm  enable_operating_limits=0  operating_limit_action=2  max_working_current=1 A  power_rating=1 W  enable_faults=0  fault_action=1  lambdaPercent=50  k_faulted=0.9999  turnsShort=0  openCct=0  groundShort=0  groundShortG=0 1/Ohm  tau_fault=1e-3 s  enable_temporal_fault=0  t_fault=1 s  enable_behavioral_fault=0  max_permissible_voltage=100 V  n_fail_on_voltage=1  max_permissible_current=1 A  t_fail_on_current=1 s  i_L_specify=off  i_L_priority=High  i_L=0 A  i_L_nominal_specify=off  i_L_nominal_unit=A  i_L_nominal_value=1
      settings: SourceProductName=Simscape Electronics  SourceProductBaseCode=SN
  L serie 2 : elec_lib/Passive Devices/Inductor  l=L_mg_3(2) H  L_tol=20  enable_L_tol=0  tol_distribution=1  nSigma=4  r=0 Ohm  g=1e-9 1/Ohm  enable_operating_limits=0  operating_limit_action=2  max_working_current=1 A  power_rating=1 W  enable_faults=0  fault_action=1  lambdaPercent=50  k_faulted=0.9999  turnsShort=0  openCct=0  groundShort=0  groundShortG=0 1/Ohm  tau_fault=1e-3 s  enable_temporal_fault=0  t_fault=1 s  enable_behavioral_fault=0  max_permissible_voltage=100 V  n_fail_on_voltage=1  max_permissible_current=1 A  t_fail_on_current=1 s  i_L_specify=off  i_L_priority=High  i_L=0 A  i_L_nominal_specify=off  i_L_nominal_unit=A  i_L_nominal_value=1
      settings: SourceProductName=Simscape Electronics  SourceProductBaseCode=SN
  L serie 3 : elec_lib/Passive Devices/Inductor  l=L_mg_3(3) H  L_tol=20  enable_L_tol=0  tol_distribution=1  nSigma=4  r=0 Ohm  g=1e-9 1/Ohm  enable_operating_limits=0  operating_limit_action=2  max_working_current=1 A  power_rating=1 W  enable_faults=0  fault_action=1  lambdaPercent=50  k_faulted=0.9999  turnsShort=0  openCct=0  groundShort=0  groundShortG=0 1/Ohm  tau_fault=1e-3 s  enable_temporal_fault=0  t_fault=1 s  enable_behavioral_fault=0  max_permissible_voltage=100 V  n_fail_on_voltage=1  max_permissible_current=1 A  t_fail_on_current=1 s  i_L_specify=off  i_L_priority=High  i_L=0 A  i_L_nominal_specify=off  i_L_nominal_unit=A  i_L_nominal_value=1
      settings: SourceProductName=Simscape Electronics  SourceProductBaseCode=SN
  L serie 4 : elec_lib/Passive Devices/Inductor  l=L_mg_3(4) H  L_tol=20  enable_L_tol=0  tol_distribution=1  nSigma=4  r=0 Ohm  g=1e-9 1/Ohm  enable_operating_limits=0  operating_limit_action=2  max_working_current=1 A  power_rating=1 W  enable_faults=0  fault_action=1  lambdaPercent=50  k_faulted=0.9999  turnsShort=0  openCct=0  groundShort=0  groundShortG=0 1/Ohm  tau_fault=1e-3 s  enable_temporal_fault=0  t_fault=1 s  enable_behavioral_fault=0  max_permissible_voltage=100 V  n_fail_on_voltage=1  max_permissible_current=1 A  t_fail_on_current=1 s  i_L_specify=off  i_L_priority=High  i_L=0 A  i_L_nominal_specify=off  i_L_nominal_unit=A  i_L_nominal_value=1
      settings: SourceProductName=Simscape Electronics  SourceProductBaseCode=SN
  L serie 5 : elec_lib/Passive Devices/Inductor  l=L_mg_3(1) H  L_tol=20  enable_L_tol=0  tol_distribution=1  nSigma=4  r=0 Ohm  g=1e-9 1/Ohm  enable_operating_limits=0  operating_limit_action=2  max_working_current=1 A  power_rating=1 W  enable_faults=0  fault_action=1  lambdaPercent=50  k_faulted=0.9999  turnsShort=0  openCct=0  groundShort=0  groundShortG=0 1/Ohm  tau_fault=1e-3 s  enable_temporal_fault=0  t_fault=1 s  enable_behavioral_fault=0  max_permissible_voltage=100 V  n_fail_on_voltage=1  max_permissible_current=1 A  t_fail_on_current=1 s  i_L_specify=off  i_L_priority=High  i_L=0 A  i_L_nominal_specify=off  i_L_nominal_unit=A  i_L_nominal_value=1
      settings: SourceProductName=Simscape Electronics  SourceProductBaseCode=SN
  L serie 6 : elec_lib/Passive Devices/Inductor  l=L_mg_4(2) H  L_tol=20  enable_L_tol=0  tol_distribution=1  nSigma=4  r=0 Ohm  g=1e-9 1/Ohm  enable_operating_limits=0  operating_limit_action=2  max_working_current=1 A  power_rating=1 W  enable_faults=0  fault_action=1  lambdaPercent=50  k_faulted=0.9999  turnsShort=0  openCct=0  groundShort=0  groundShortG=0 1/Ohm  tau_fault=1e-3 s  enable_temporal_fault=0  t_fault=1 s  enable_behavioral_fault=0  max_permissible_voltage=100 V  n_fail_on_voltage=1  max_permissible_current=1 A  t_fail_on_current=1 s  i_L_specify=off  i_L_priority=High  i_L=0 A  i_L_nominal_specify=off  i_L_nominal_unit=A  i_L_nominal_value=1
      settings: SourceProductName=Simscape Electronics  SourceProductBaseCode=SN
  L serie 7 : elec_lib/Passive Devices/Inductor  l=L_mg_4(3) H  L_tol=20  enable_L_tol=0  tol_distribution=1  nSigma=4  r=0 Ohm  g=1e-9 1/Ohm  enable_operating_limits=0  operating_limit_action=2  max_working_current=1 A  power_rating=1 W  enable_faults=0  fault_action=1  lambdaPercent=50  k_faulted=0.9999  turnsShort=0  openCct=0  groundShort=0  groundShortG=0 1/Ohm  tau_fault=1e-3 s  enable_temporal_fault=0  t_fault=1 s  enable_behavioral_fault=0  max_permissible_voltage=100 V  n_fail_on_voltage=1  max_permissible_current=1 A  t_fail_on_current=1 s  i_L_specify=off  i_L_priority=High  i_L=0 A  i_L_nominal_specify=off  i_L_nominal_unit=A  i_L_nominal_value=1
      settings: SourceProductName=Simscape Electronics  SourceProductBaseCode=SN
  L serie 8 : elec_lib/Passive Devices/Inductor  l=L_mg_4(4) H  L_tol=20  enable_L_tol=0  tol_distribution=1  nSigma=4  r=0 Ohm  g=1e-9 1/Ohm  enable_operating_limits=0  operating_limit_action=2  max_working_current=1 A  power_rating=1 W  enable_faults=0  fault_action=1  lambdaPercent=50  k_faulted=0.9999  turnsShort=0  openCct=0  groundShort=0  groundShortG=0 1/Ohm  tau_fault=1e-3 s  enable_temporal_fault=0  t_fault=1 s  enable_behavioral_fault=0  max_permissible_voltage=100 V  n_fail_on_voltage=1  max_permissible_current=1 A  t_fail_on_current=1 s  i_L_specify=off  i_L_priority=High  i_L=0 A  i_L_nominal_specify=off  i_L_nominal_unit=A  i_L_nominal_value=1
      settings: SourceProductName=Simscape Electronics  SourceProductBaseCode=SN
  L serie 9 : elec_lib/Passive Devices/Inductor  l=L_mg_1(1) H  L_tol=20  enable_L_tol=0  tol_distribution=1  nSigma=4  r=0 Ohm  g=1e-9 1/Ohm  enable_operating_limits=0  operating_limit_action=2  max_working_current=1 A  power_rating=1 W  enable_faults=0  fault_action=1  lambdaPercent=50  k_faulted=0.9999  turnsShort=0  openCct=0  groundShort=0  groundShortG=0 1/Ohm  tau_fault=1e-3 s  enable_temporal_fault=0  t_fault=1 s  enable_behavioral_fault=0  max_permissible_voltage=100 V  n_fail_on_voltage=1  max_permissible_current=1 A  t_fail_on_current=1 s  i_L_specify=off  i_L_priority=High  i_L=0 A  i_L_nominal_specify=off  i_L_nominal_unit=A  i_L_nominal_value=1
      settings: SourceProductName=Simscape Electronics  SourceProductBaseCode=SN
  MATLAB Function1 : MATLAB Function  TreatAsAtomicUnit=on
  MATLAB Function2 : MATLAB Function  TreatAsAtomicUnit=on
  MATLAB Function3 : MATLAB Function  TreatAsAtomicUnit=on
  MATLAB Function4 : MATLAB Function  TreatAsAtomicUnit=on
  MATLAB Function5 : MATLAB Function  TreatAsAtomicUnit=on
  Manual Switch{1..17} (17 alike) : ManualSwitch  CurrentSetting=0
  Mux{,2,4,6..7,12..13} (7 alike) : Mux
  Mux1 : Mux  Inputs=5
  Mux10 : Mux  Inputs=3
  Mux11 : Mux  Inputs=2
  Mux14 : Mux  Inputs=5
  Mux3 : Mux  Inputs=5
  Mux5 : Mux  Inputs=3
  Mux8 : Mux  Inputs=3
  Mux9 : Mux  Inputs=2
  PI i 1 : TransferFcn  Numerator=[k_pi_4 k_ii_4 ]  Denominator=[1 0]
  PI i 2 : TransferFcn  Numerator=[k_pi_1 k_ii_1 ]  Denominator=[1 0]
  PI i 3 : TransferFcn  Numerator=[k_pi_3 k_ii_3 ]  Denominator=[1 0]
  PI i 4 : TransferFcn  Numerator=[k_pi_2 k_ii_2 ]  Denominator=[1 0]
  PI i1 : TransferFcn  Numerator=[k_pi_3 k_ii_3 ]  Denominator=[1 0]
  PI i2 : TransferFcn  Numerator=[k_pi_4 k_ii_4 ]  Denominator=[1 0]
  PI i3 : TransferFcn  Numerator=[k_pi_4 k_ii_4]  Denominator=[1 0]
  PI i4 : TransferFcn  Numerator=[k_pi_3 k_ii_3]  Denominator=[1 0]
  PI i5 : TransferFcn  Numerator=[k_pi_3 k_ii_3 ]  Denominator=[1 0]
  PI i6 : TransferFcn  Numerator=[k_pi_4 k_ii_4 ]  Denominator=[1 0]
  PI i7 : TransferFcn  Numerator=[k_pi_2 k_ii_2]  Denominator=[1 0]
  PI i8 : TransferFcn  Numerator=[k_pi_1 k_ii_1]  Denominator=[1 0]
  PI i9 : TransferFcn  Numerator=[k_pi_1 k_ii_1 ]  Denominator=[1 0]
  PS-Simulink Converter{,1..55,60..62} (59 alike) : nesl_utility/PS-Simulink Converter  PhysicalDomain=network_engine_domain  SubClassName=ps_output  LeftPortType=input  RightPortType=output  PseudoPeriodic=off  Frequencies=[]  Unit=1  AffineConversion=off
  Product{1..4} (4 alike) : Product  Commented=on
  Product5 : Product
  Product6 : Product
  R serie 1 : fl_lib/Electrical/Electrical Elements/Resistor  R=rd_mg_3(1) Ohm  i_specify=off  i_priority=None  i=0 A  i_nominal_specify=off  i_nominal_unit=A  i_nominal_value=1  v_specify=off  v_priority=None  v=0 V  v_nominal_specify=off  v_nominal_unit=V  v_nominal_value=1
  R serie 10 : fl_lib/Electrical/Electrical Elements/Resistor  R=rd_mg_4(2) Ohm  i_specify=off  i_priority=None  i=0 A  i_nominal_specify=off  i_nominal_unit=A  i_nominal_value=1  v_specify=off  v_priority=None  v=0 V  v_nominal_specify=off  v_nominal_unit=V  v_nominal_value=1
  R serie 11 : fl_lib/Electrical/Electrical Elements/Resistor  R=rd_mg_4(3) Ohm  i_specify=off  i_priority=None  i=0 A  i_nominal_specify=off  i_nominal_unit=A  i_nominal_value=1  v_specify=off  v_priority=None  v=0 V  v_nominal_specify=off  v_nominal_unit=V  v_nominal_value=1
  R serie 12 : fl_lib/Electrical/Electrical Elements/Resistor  R=1/(g12_3) Ohm  i_specify=off  i_priority=None  i=0 A  i_nominal_specify=off  i_nominal_unit=A  i_nominal_value=1  v_specify=off  v_priority=None  v=0 V  v_nominal_specify=off  v_nominal_unit=V  v_nominal_value=1
  R serie 13 : fl_lib/Electrical/Electrical Elements/Resistor  R=1/(g13_3) Ohm  i_specify=off  i_priority=None  i=0 A  i_nominal_specify=off  i_nominal_unit=A  i_nominal_value=1  v_specify=off  v_priority=None  v=0 V  v_nominal_specify=off  v_nominal_unit=V  v_nominal_value=1
  R serie 14 : fl_lib/Electrical/Electrical Elements/Resistor  R=rd_mg_4(4) Ohm  i_specify=off  i_priority=None  i=0 A  i_nominal_specify=off  i_nominal_unit=A  i_nominal_value=1  v_specify=off  v_priority=None  v=0 V  v_nominal_specify=off  v_nominal_unit=V  v_nominal_value=1
  R serie 15 : fl_lib/Electrical/Electrical Elements/Resistor  R=1/(g24_4) Ohm  i_specify=off  i_priority=None  i=0 A  i_nominal_specify=off  i_nominal_unit=A  i_nominal_value=1  v_specify=off  v_priority=None  v=0 V  v_nominal_specify=off  v_nominal_unit=V  v_nominal_value=1
  R serie 16 : fl_lib/Electrical/Electrical Elements/Resistor  R=1/(g34_4) Ohm  i_specify=off  i_priority=None  i=0 A  i_nominal_specify=off  i_nominal_unit=A  i_nominal_value=1  v_specify=off  v_priority=None  v=0 V  v_nominal_specify=off  v_nominal_unit=V  v_nominal_value=1
  R serie 17 : fl_lib/Electrical/Electrical Elements/Resistor  R=1/(g23_4) Ohm  i_specify=off  i_priority=None  i=0 A  i_nominal_specify=off  i_nominal_unit=A  i_nominal_value=1  v_specify=off  v_priority=None  v=0 V  v_nominal_specify=off  v_nominal_unit=V  v_nominal_value=1
  R serie 18 : fl_lib/Electrical/Electrical Elements/Resistor  R=1/g34 Ohm  i_specify=off  i_priority=None  i=0 A  i_nominal_specify=off  i_nominal_unit=A  i_nominal_value=1  v_specify=off  v_priority=None  v=0 V  v_nominal_specify=off  v_nominal_unit=V  v_nominal_value=1
  R serie 19 : fl_lib/Electrical/Electrical Elements/Resistor  R=rd_mg_1(1) Ohm  i_specify=off  i_priority=None  i=0 A  i_nominal_specify=off  i_nominal_unit=A  i_nominal_value=1  v_specify=off  v_priority=None  v=0 V  v_nominal_specify=off  v_nominal_unit=V  v_nominal_value=1
  R serie 2 : fl_lib/Electrical/Electrical Elements/Resistor  R=rd_mg_3(2) Ohm  i_specify=off  i_priority=None  i=0 A  i_nominal_specify=off  i_nominal_unit=A  i_nominal_value=1  v_specify=off  v_priority=None  v=0 V  v_nominal_specify=off  v_nominal_unit=V  v_nominal_value=1
  R serie 20 : fl_lib/Electrical/Electrical Elements/Resistor  R=1/(g12_1) Ohm  i_specify=off  i_priority=None  i=0 A  i_nominal_specify=off  i_nominal_unit=A  i_nominal_value=1  v_specify=off  v_priority=None  v=0 V  v_nominal_specify=off  v_nominal_unit=V  v_nominal_value=1
  R serie 21 : fl_lib/Electrical/Electrical Elements/Resistor  R=1/(g13_1) Ohm  i_specify=off  i_priority=None  i=0 A  i_nominal_specify=off  i_nominal_unit=A  i_nominal_value=1  v_specify=off  v_priority=None  v=0 V  v_nominal_specify=off  v_nominal_unit=V  v_nominal_value=1
  R serie 22 : fl_lib/Electrical/Electrical Elements/Resistor  R=rd_mg_1(2) Ohm  i_specify=off  i_priority=None  i=0 A  i_nominal_specify=off  i_nominal_unit=A  i_nominal_value=1  v_specify=off  v_priority=None  v=0 V  v_nominal_specify=off  v_nominal_unit=V  v_nominal_value=1
  R serie 23 : fl_lib/Electrical/Electrical Elements/Resistor  R=rd_mg_1(3) Ohm  i_specify=off  i_priority=None  i=0 A  i_nominal_specify=off  i_nominal_unit=A  i_nominal_value=1  v_specify=off  v_priority=None  v=0 V  v_nominal_specify=off  v_nominal_unit=V  v_nominal_value=1
  R serie 24 : fl_lib/Electrical/Electrical Elements/Resistor  R=rd_mg_2(1) Ohm  i_specify=off  i_priority=None  i=0 A  i_nominal_specify=off  i_nominal_unit=A  i_nominal_value=1  v_specify=off  v_priority=None  v=0 V  v_nominal_specify=off  v_nominal_unit=V  v_nominal_value=1
  R serie 25 : fl_lib/Electrical/Electrical Elements/Resistor  R=1/(g12_2) Ohm  i_specify=off  i_priority=None  i=0 A  i_nominal_specify=off  i_nominal_unit=A  i_nominal_value=1  v_specify=off  v_priority=None  v=0 V  v_nominal_specify=off  v_nominal_unit=V  v_nominal_value=1
  R serie 26 : fl_lib/Electrical/Electrical Elements/Resistor  R=1/(g23_1) Ohm  i_specify=off  i_priority=None  i=0 A  i_nominal_specify=off  i_nominal_unit=A  i_nominal_value=1  v_specify=off  v_priority=None  v=0 V  v_nominal_specify=off  v_nominal_unit=V  v_nominal_value=1
  R serie 27 : fl_lib/Electrical/Electrical Elements/Resistor  R=1/g12 Ohm  i_specify=off  i_priority=None  i=0 A  i_nominal_specify=off  i_nominal_unit=A  i_nominal_value=1  v_specify=off  v_priority=None  v=0 V  v_nominal_specify=off  v_nominal_unit=V  v_nominal_value=1
  R serie 28 : fl_lib/Electrical/Electrical Elements/Resistor  R=rd_mg_2(2) Ohm  i_specify=off  i_priority=None  i=0 A  i_nominal_specify=off  i_nominal_unit=A  i_nominal_value=1  v_specify=off  v_priority=None  v=0 V  v_nominal_specify=off  v_nominal_unit=V  v_nominal_value=1
  R serie 29 : fl_lib/Electrical/Electrical Elements/Resistor  R=1/g24 Ohm  i_specify=off  i_priority=None  i=0 A  i_nominal_specify=off  i_nominal_unit=A  i_nominal_value=1  v_specify=off  v_priority=None  v=0 V  v_nominal_specify=off  v_nominal_unit=V  v_nominal_value=1
  R serie 3 : fl_lib/Electrical/Electrical Elements/Resistor  R=rd_mg_3(3) Ohm  i_specify=off  i_priority=None  i=0 A  i_nominal_specify=off  i_nominal_unit=A  i_nominal_value=1  v_specify=off  v_priority=None  v=0 V  v_nominal_specify=off  v_nominal_unit=V  v_nominal_value=1
  R serie 30 : fl_lib/Electrical/Electrical Elements/Resistor  R=1/g13 Ohm  i_specify=off  i_priority=None  i=0 A  i_nominal_specify=off  i_nominal_unit=A  i_nominal_value=1  v_specify=off  v_priority=None  v=0 V  v_nominal_specify=off  v_nominal_unit=V  v_nominal_value=1
  R serie 4 : fl_lib/Electrical/Electrical Elements/Resistor  R=rd_mg_3(4) Ohm  i_specify=off  i_priority=None  i=0 A  i_nominal_specify=off  i_nominal_unit=A  i_nominal_value=1  v_specify=off  v_priority=None  v=0 V  v_nominal_specify=off  v_nominal_unit=V  v_nominal_value=1
  R serie 5 : fl_lib/Electrical/Electrical Elements/Resistor  R=1/(g24_3) Ohm  i_specify=off  i_priority=None  i=0 A  i_nominal_specify=off  i_nominal_unit=A  i_nominal_value=1  v_specify=off  v_priority=None  v=0 V  v_nominal_specify=off  v_nominal_unit=V  v_nominal_value=1
  R serie 6 : fl_lib/Electrical/Electrical Elements/Resistor  R=1/(g34_3) Ohm  i_specify=off  i_priority=None  i=0 A  i_nominal_specify=off  i_nominal_unit=A  i_nominal_value=1  v_specify=off  v_priority=None  v=0 V  v_nominal_specify=off  v_nominal_unit=V  v_nominal_value=1
  R serie 7 : fl_lib/Electrical/Electrical Elements/Resistor  R=rd_mg_3(1) Ohm  i_specify=off  i_priority=None  i=0 A  i_nominal_specify=off  i_nominal_unit=A  i_nominal_value=1  v_specify=off  v_priority=None  v=0 V  v_nominal_specify=off  v_nominal_unit=V  v_nominal_value=1
  R serie 8 : fl_lib/Electrical/Electrical Elements/Resistor  R=1/(g12_4) Ohm  i_specify=off  i_priority=None  i=0 A  i_nominal_specify=off  i_nominal_unit=A  i_nominal_value=1  v_specify=off  v_priority=None  v=0 V  v_nominal_specify=off  v_nominal_unit=V  v_nominal_value=1
  R serie 9 : fl_lib/Electrical/Electrical Elements/Resistor  R=1/(g13_4) Ohm  i_specify=off  i_priority=None  i=0 A  i_nominal_specify=off  i_nominal_unit=A  i_nominal_value=1  v_specify=off  v_priority=None  v=0 V  v_nominal_specify=off  v_nominal_unit=V  v_nominal_value=1
  Saturation{1..51} (51 alike) : Saturate  UpperLimit=100  LowerLimit=-100
  Scope{,9,48..49,92} (5 alike) : Scope  NumInputPorts=2
  Scope1 : Scope  Commented=on
  Scope{2..8,10..15,17..47,50..91,93..95} (89 alike) : Scope
  Scope16 : Scope  Commented=on
  Simulink-PS Converter{,1..20,22..24,26..27} (26 alike) : nesl_utility/Simulink-PS Converter  PhysicalDomain=network_engine_domain  SubClassName=ps_input  LeftPortType=input  RightPortType=output  PseudoPeriodic=off  Frequencies=[]  NoiseDistribution=none  NoiseParameters=[]  Unit=1  AffineConversion=off  FilteringAndDerivatives=provide  SimscapeFilterOrder=1  InputFilterTimeConstant=0.001  UdotUserProvided=0
  Sine Wave{1..4} (4 alike) : Sin  Commented=on  Amplitude=tau/2  Frequency=h*2*3.14  SampleTime=0
  Sine Wave5 : Sin  Amplitude=tau/4  Bias=tau/4  Frequency=h*2*3.14  SampleTime=0
  Sine Wave6 : Sin  Amplitude=tau/4  Bias=tau/4  Frequency=h*2*3.14  SampleTime=0
  Solver Configuration : nesl_utility/Solver Configuration  PhysicalDomain=network_engine_domain  SubClassName=solver  LeftPortType=input  RightPortType=generic  Tones=[]  Harmonics=[]  SimulateNoise=off  Profile=off  UseLocalSampling=off  EnableSwitchedLinearOptims=on  FrequencyDomain=off  UseCCode=off  RelTol=0.001  AbsTol=1e-06  MinStep=1e-09  ToWorkspace=off  RevertToSquareIcSolve=off  NumHomotopyIterations=100  PhasorMode=off  PhasorModeNumHarmonics=1  DoDC=off  ResidualTolerance=1e-09  UseLocalSolver=off  LocalSolverChoice=NE_BACKWARD_EULER_ADVANCER  LocalSolverSampleTime=0.001  DoFixedCost=off  MaxNonlinIter=3  MaxModeIter=2  LinearAlgebra=Sparse  EquationFormulation=NE_TIME_EF  DelaysMemoryBudget=1024  AutomaticFiltering=on  FilteringTimeConstant=0.001
  Solver Configuration1 : nesl_utility/Solver Configuration  Commented=on  PhysicalDomain=network_engine_domain  SubClassName=solver  LeftPortType=input  RightPortType=generic  Tones=[]  Harmonics=[]  SimulateNoise=off  Profile=off  UseLocalSampling=off  EnableSwitchedLinearOptims=on  FrequencyDomain=off  UseCCode=off  RelTol=0.001  AbsTol=1e-06  MinStep=1e-09  ToWorkspace=off  RevertToSquareIcSolve=off  NumHomotopyIterations=100  PhasorMode=off  PhasorModeNumHarmonics=1  DoDC=off  ResidualTolerance=1e-09  UseLocalSolver=off  LocalSolverChoice=NE_BACKWARD_EULER_ADVANCER  LocalSolverSampleTime=0.001  DoFixedCost=off  MaxNonlinIter=3  MaxModeIter=2  LinearAlgebra=Sparse  EquationFormulation=NE_TIME_EF  DelaysMemoryBudget=1024  AutomaticFiltering=on  FilteringTimeConstant=0.001
  Solver Configuration2 : nesl_utility/Solver Configuration  Commented=on  PhysicalDomain=network_engine_domain  SubClassName=solver  LeftPortType=input  RightPortType=generic  Tones=[]  Harmonics=[]  SimulateNoise=off  Profile=off  UseLocalSampling=off  EnableSwitchedLinearOptims=on  FrequencyDomain=off  UseCCode=off  RelTol=0.001  AbsTol=1e-06  MinStep=1e-09  ToWorkspace=off  RevertToSquareIcSolve=off  NumHomotopyIterations=100  PhasorMode=off  PhasorModeNumHarmonics=1  DoDC=off  ResidualTolerance=1e-09  UseLocalSolver=off  LocalSolverChoice=NE_BACKWARD_EULER_ADVANCER  LocalSolverSampleTime=0.001  DoFixedCost=off  MaxNonlinIter=3  MaxModeIter=2  LinearAlgebra=Sparse  EquationFormulation=NE_TIME_EF  DelaysMemoryBudget=1024  AutomaticFiltering=on  FilteringTimeConstant=0.001
  Solver Configuration3 : nesl_utility/Solver Configuration  Commented=on  PhysicalDomain=network_engine_domain  SubClassName=solver  LeftPortType=input  RightPortType=generic  Tones=[]  Harmonics=[]  SimulateNoise=off  Profile=off  UseLocalSampling=off  EnableSwitchedLinearOptims=on  FrequencyDomain=off  UseCCode=off  RelTol=0.001  AbsTol=1e-06  MinStep=1e-09  ToWorkspace=off  RevertToSquareIcSolve=off  NumHomotopyIterations=100  PhasorMode=off  PhasorModeNumHarmonics=1  DoDC=off  ResidualTolerance=1e-09  UseLocalSolver=off  LocalSolverChoice=NE_BACKWARD_EULER_ADVANCER  LocalSolverSampleTime=0.001  DoFixedCost=off  MaxNonlinIter=3  MaxModeIter=2  LinearAlgebra=Sparse  EquationFormulation=NE_TIME_EF  DelaysMemoryBudget=1024  AutomaticFiltering=on  FilteringTimeConstant=0.001
  Step{1,12,37,39} (4 alike) : Step  Commented=on  Time=5  SampleTime=0
  Step10 : Step  Time=time_2  After=P_load_vertex_3(1,1)  SampleTime=0
  Step{11,14,24,26..28,32,35,45,47..48,52,58,60..61,65..66} (17 alike) : Step  Time=0  SampleTime=0
  Step13 : Step  Time=time_2  After=P_load_vertex_4(1,1)  SampleTime=0
  Step15 : Step  Time=time_1  After=P_load_vertex_3(16,3)  SampleTime=0
  Step16 : Step  Time=time_4  After=P_load_vertex_3(16,3)  SampleTime=0
  Step{17,21,42,55} (4 alike) : Step  Commented=on  Time=50  After=-100  SampleTime=0
  Step18 : Step  Time=time_2  After=P_load_vertex_3(1,3)  SampleTime=0
  Step19 : Step  Time=time_1  After=P_load_vertex_4(16,3)  SampleTime=0
  Step2 : Step  Time=time_1  After=P_load_vertex_3(16,2)  SampleTime=0
  Step20 : Step  Time=time_4  After=P_load_vertex_4(16,3)  SampleTime=0
  Step22 : Step  Time=time_2  After=P_load_vertex_4(1,3)  SampleTime=0
  Step23 : Step  Time=time_1  After=P_load_vertex_4(16,2)  SampleTime=0
  Step25 : Step  Time=time_4  After=P_load_vertex_4(16,2)  SampleTime=0
  Step29 : Step  Time=time_2  After=P_load_vertex_4(1,2)  SampleTime=0
  Step3 : Step  Time=time_4  After=P_load_vertex_3(16,2)  SampleTime=0
  Step30 : Step  Time=time_1  After=P_load_vertex_4(16,4)  SampleTime=0
  Step31 : Step  Time=time_1  After=P_load_vertex_4(16,1)  SampleTime=0
  Step33 : Step  Time=time_4  After=P_load_vertex_4(16,4)  SampleTime=0
  Step34 : Step  Time=time_4  After=P_load_vertex_4(16,1)  SampleTime=0
  Step36 : Step  Time=time_2  After=P_load_vertex_4(1,4)  SampleTime=0
  Step38 : Step  Time=time_2  After=P_load_vertex_1(1,1)  SampleTime=0
  Step4 : Step  Time=time_2  After=P_load_vertex_3(1,2)  SampleTime=0
  Step40 : Step  Time=time_1  After=P_load_vertex_1(8,3)  SampleTime=0
  Step41 : Step  Time=time_4  After=P_load_vertex_1(8,3)  SampleTime=0
  Step43 : Step  Time=time_2  After=P_load_vertex_1(1,3)  SampleTime=0
  Step44 : Step  Time=time_1  After=P_load_vertex_1(8,2)  SampleTime=0
  Step46 : Step  Time=time_4  After=P_load_vertex_1(8,2)  SampleTime=0
  Step49 : Step  Time=time_2  After=P_load_vertex_1(8,2)  SampleTime=0
  Step5 : Step  Time=time_1  After=P_load_vertex_3(16,4)  SampleTime=0
  Step50 : Step  Time=time_2  After=P_load_vertex_2(1,1)  SampleTime=0
  Step51 : Step  Time=time_1  After=P_load_vertex_1(8,1)  SampleTime=0
  Step53 : Step  Time=time_4  After=P_load_vertex_1(8,1)  SampleTime=0
  Step54 : Step  Time=time_1  SampleTime=0
  Step56 : Step  Time=time_2  After=-100  SampleTime=0
  Step57 : Step  Time=time_1  After=P_load_vertex_2(4,2)  SampleTime=0
  Step59 : Step  Time=time_4  After=P_load_vertex_2(4,2)  SampleTime=0
  Step6 : Step  Time=time_1  After=P_load_vertex_3(16,1)  SampleTime=0
  Step62 : Step  Time=time_2  After=P_load_vertex_2(1,2)  SampleTime=0
  Step63 : Step  Time=time_1  After=P_load_vertex_2(4,1)  SampleTime=0
  Step64 : Step  Time=time_4  After=P_load_vertex_2(4,1)  SampleTime=0
  Step67 : Step  Time=time_7  After=-0.9 *P_load_vertex_1(1,1)  SampleTime=0
  Step68 : Step  Time=time_a_up  After=4  SampleTime=0
  Step69 : Step  Time=time_a_down  After=-9  SampleTime=0
  Step7 : Step  Time=time_4  After=P_load_vertex_3(16,4)  SampleTime=0
  Step70 : Step  Time=time_6  After=3  SampleTime=0
  Step71 : Step  Time=time_1  SampleTime=0
  Step72 : Step  Time=time_6  After=3  SampleTime=0
  Step73 : Step  Time=time_7  After=-0.9 *P_load_vertex_1(1,2)  SampleTime=0
  Step74 : Step  Time=time_7  After=-0.9 *P_load_vertex_1(1,3)  SampleTime=0
  Step75 : Step  Time=time_7  After=-0.9 *P_load_vertex_2(1,1)  SampleTime=0
  Step76 : Step  Time=time_7  After=-0.9 *P_load_vertex_2(1,2)  SampleTime=0
  Step77 : Step  Time=time_7  After=-0.9 * P_load_vertex_3(1,1)  SampleTime=0
  Step78 : Step  Time=time_7  After=-0.9 * P_load_vertex_3(1,2)  SampleTime=0
  Step79 : Step  Time=time_7  After=-0.9 * P_load_vertex_3(1,4)  SampleTime=0
  Step8 : Step  Time=time_4  After=P_load_vertex_3(16,1)  SampleTime=0
  Step80 : Step  Time=time_7  After=-0.9 * P_load_vertex_3(1,3)  SampleTime=0
  Step81 : Step  Time=time_7  After=-0.9 * P_load_vertex_4(1,4)  SampleTime=0
  Step82 : Step  Time=time_7  After=-0.9 * P_load_vertex_4(1,3)  SampleTime=0
  Step83 : Step  Time=time_7  After=-0.9 * P_load_vertex_4(1,2)  SampleTime=0
  Step84 : Step  Time=time_7  After=-0.9 * P_load_vertex_4(1,1)  SampleTime=0
  Step85 : Step  Time=time_tau_down  After=-3  SampleTime=0
  Step86 : Step  Time=time_tau_down  After=-3  SampleTime=0
  Step9 : Step  Time=time_2  After=P_load_vertex_3(1,4)  SampleTime=0
  Subsystem : Subsystem
  Subsystem1 : Subsystem
  Subsystem2 : Subsystem
  Subsystem3 : Subsystem
  Sum{1..2,4..6,8,10,12..14,16..17,19..21,23,25..26,28..33,35,37,39,41,43..44,46..47,49..50} (34 alike) : Sum  Inputs=+-|
  Sum{3,7,9,11,15,18,22,24,27,34,36,38,40,42,45,48,51} (17 alike) : Sum  Inputs=++|
  Switch{1..17} (17 alike) : Switch  Criteria=u2 > Threshold
  To Workspace : ToWorkspace  VariableName=i_1_sa  SaveFormat=Timeseries  SampleTime=-1
  To Workspace1 : ToWorkspace  VariableName=i_2_sa  SaveFormat=Timeseries  SampleTime=-1
  To Workspace10 : ToWorkspace  VariableName=i_4_sa  SaveFormat=Timeseries  SampleTime=-1
  To Workspace11 : ToWorkspace  VariableName=deltaR4_sa1  SaveFormat=Timeseries  SampleTime=-1
  To Workspace12 : ToWorkspace  VariableName=V_MG_sa1  SaveFormat=Timeseries  SampleTime=-1
  To Workspace13 : ToWorkspace  VariableName=i_1_sa2  SaveFormat=Timeseries  SampleTime=-1
  To Workspace14 : ToWorkspace  VariableName=i_2_sa2  SaveFormat=Timeseries  SampleTime=-1
  To Workspace15 : ToWorkspace  VariableName=deltaR1_sa1  SaveFormat=Timeseries  SampleTime=-1
  To Workspace16 : ToWorkspace  VariableName=deltaR2_sa1  SaveFormat=Timeseries  SampleTime=-1
  To Workspace17 : ToWorkspace  VariableName=deltaR3_sa1  SaveFormat=Timeseries  SampleTime=-1
  To Workspace18 : ToWorkspace  VariableName=i_1_sa3  SaveFormat=Timeseries  SampleTime=-1
  To Workspace19 : ToWorkspace  VariableName=i_2_sa3  SaveFormat=Timeseries  SampleTime=-1
  To Workspace2 : ToWorkspace  VariableName=i_1_sa1  SaveFormat=Timeseries  SampleTime=-1
  To Workspace20 : ToWorkspace  VariableName=deltaR1_sa2  SaveFormat=Timeseries  SampleTime=-1
  To Workspace21 : ToWorkspace  VariableName=deltaR2_sa2  SaveFormat=Timeseries  SampleTime=-1
  To Workspace22 : ToWorkspace  VariableName=deltaR3_sa2  SaveFormat=Timeseries  SampleTime=-1
  To Workspace23 : ToWorkspace  VariableName=V_MG_sa2  SaveFormat=Timeseries  SampleTime=-1
  To Workspace24 : ToWorkspace  VariableName=deltaR1_sa3  SaveFormat=Timeseries  SampleTime=-1
  To Workspace25 : ToWorkspace  VariableName=deltaR2_sa3  SaveFormat=Timeseries  SampleTime=-1
  To Workspace26 : ToWorkspace  VariableName=deltaR1_sa4  SaveFormat=Timeseries  SampleTime=-1
  To Workspace27 : ToWorkspace  VariableName=V_MG_sa3  SaveFormat=Timeseries  SampleTime=-1
  To Workspace28 : ToWorkspace  VariableName=V_MG_sa4  SaveFormat=Timeseries  SampleTime=-1
  To Workspace29 : ToWorkspace  VariableName=deltaR1_sa5  SaveFormat=Timeseries  SampleTime=-1
  To Workspace3 : ToWorkspace  VariableName=i_2_sa1  SaveFormat=Timeseries  SampleTime=-1
  To Workspace30 : ToWorkspace  VariableName=deltaR1_sa6  SaveFormat=Timeseries  SampleTime=-1
  To Workspace31 : ToWorkspace  VariableName=deltaR1_sa7  SaveFormat=Timeseries  SampleTime=-1
  To Workspace32 : ToWorkspace  VariableName=I_MG_2  SaveFormat=Timeseries  SampleTime=-1
  To Workspace33 : ToWorkspace  VariableName=I_MG_1  SaveFormat=Timeseries  SampleTime=-1
  To Workspace34 : ToWorkspace  VariableName=I_MG_4  SaveFormat=Timeseries  SampleTime=-1
  To Workspace35 : ToWorkspace  VariableName=I_MG_3  SaveFormat=Timeseries  SampleTime=-1
  To Workspace4 : ToWorkspace  VariableName=deltaR1_sa  SaveFormat=Timeseries  SampleTime=-1
  To Workspace5 : ToWorkspace  VariableName=deltaR2_sa  SaveFormat=Timeseries  SampleTime=-1
  To Workspace6 : ToWorkspace  VariableName=i_4_sa1  SaveFormat=Timeseries  SampleTime=-1
  To Workspace7 : ToWorkspace  VariableName=deltaR4_sa  SaveFormat=Timeseries  SampleTime=-1
  To Workspace8 : ToWorkspace  VariableName=deltaR3_sa  SaveFormat=Timeseries  SampleTime=-1
  To Workspace9 : ToWorkspace  VariableName=V_MG_sa  SaveFormat=Timeseries  SampleTime=-1
  Variable Time Delay : VariableTransportDelay  MaximumDelay=10
  Variable Time Delay1 : VariableTransportDelay  MaximumDelay=10
  Voltage bus {1..12,14} (13 alike) : fl_lib/Electrical/Electrical Sensors/Voltage Sensor
  Voltage output {1..12,14} (13 alike) : fl_lib/Electrical/Electrical Sensors/Voltage Sensor
  wires:
  Constant14/1 -> Switch15/3
  MATLAB Function1/3(error_3) -> [error_i_3_3]
  [V_REF_c] -> Add44/2
  Add51/1 -> [delta_I_2_3]
  Gain15/1 -> Add51/2
  Switch16/1 -> Add51/1
  Close loop equivalent25/1 -> Manual Switch16/1
  [delta_V_2_3] -> Add50/3
  Constant22/1 -> Manual Switch17/2
  [V_ref_tot_2_3] -> Add49/2
  Add39/1 -> [V_ref_tot_3_3]
  Constant13/1 -> Switch16/3
  Manual Switch17/1 -> Add49/1
  Sum9/1 -> Sum8/2, [i_prom_1_3]
  Saturation8/1 -> PI i5/1, Scope27/1
  Sum10/1 -> Saturation8/1
  Saturation12/1 -> Mux7/2
  Saturation13/1 -> Mux7/1
  Step35/1 -> Switch16/2
  PI i5/1 -> Switch17/1, To Workspace22/1, Scope29/1
  Manual Switch13/1 -> Add33/1
  [i_prom_1_3] -> Saturation13/1
  Switch17/1 -> Add42/1
  [io_source_3_3] -> Gain13/1
  Sum11/1 -> Sum10/2, Scope5/1, [i_prom_3_3]
  [io_source_2_3] -> Gain15/1
  Add49/1 -> [V_out_source_2_3]
  Add45/1 -> [delta_I_1_3]
  [error_i_1_3] -> Integrator4/1
  Sum6/1 -> Saturation10/1
  [i_prom_2_3] -> Saturation12/1
  Step28/1 -> Switch17/2
  Constant21/1 -> Manual Switch16/2
  Constant20/1 -> Switch17/3
  [delta_V_3_3] -> Add39/3
  [error_i_3_3] -> Integrator5/1
  Manual Switch16/1 -> Add31/1
  [V_REF_c] -> Add50/2
  Saturation10/1 -> PI i 3/1, Scope23/1
  Integrator5/1 -> Sum11/2
  [io_source_1_3] -> Gain18/1
  Saturation11/1 -> Mux7/3
  Saturation5/1 -> Close loop equivalent1/1
  Saturation4/1 -> Close loop equivalent2/1
  [V_ref_tot_3_3] -> Add31/2
  Saturation9/1 -> PI i4/1, Scope21/1
  [delta_V_1_3] -> Add44/3
  MATLAB Function1/2(error_2) -> [error_i_2_3]
  Saturation6/1 -> Close loop equivalent3/1
  Sum7/1 -> [i_prom_2_3], Sum6/2
  Sum8/1 -> Saturation9/1
  Gain12/1 -> Sum6/1, Sum7/1
  Integrator4/1 -> Sum9/2
  Close loop equivalent23/1 -> Manual Switch13/1
  [i_prom_3_3] -> Saturation11/1
  MATLAB Function1/1(error_1) -> [error_i_1_3]
  Close loop equivalent22/1 -> Manual Switch17/1
  Add31/1 -> [V_out_source_3_3]
  From104/1 -> Close loop equivalent22/1
  Gain16/1 -> Add42/2
  PI i4/1 -> To Workspace20/1, Scope22/1, Switch15/1
  [delta_I_3_3] -> Add39/1
  From113/1 -> Close loop equivalent23/1
  [V_REF_c] -> Add39/2
  Switch15/1 -> Add45/1
  Add50/1 -> [V_ref_tot_2_3]
  Gain13/1 -> Sum11/1, Sum10/1
  [delta_I_1_3] -> Add44/1
  Add33/1 -> [V_out_source_1_3]
  Close loop equivalent2/1 -> Scope26/1, [delta_V_2_3]
  Mux7/1 -> MATLAB Function1/1(i)
  Integrator3/1 -> Sum7/2
  [io_source_3_3] -> Gain16/1
  [error_i_2_3] -> Integrator3/1
  Step32/1 -> Switch15/2
  Constant19/1 -> Manual Switch13/2
  Add42/1 -> [delta_I_3_3]
  [io_source_2_3] -> Gain12/1
  Close loop equivalent3/1 -> Scope25/1, [delta_V_1_3]
  Gain17/1 -> Sum9/1, Sum8/1
  Gain18/1 -> Add45/2
  PI i 3/1 -> To Workspace21/1, Scope24/1, Switch16/1
  [io_source_1_3] -> Gain17/1
  [delta_I_2_3] -> Add50/1
  Add44/1 -> [V_ref_tot_1_3]
  From116/1 -> Close loop equivalent25/1
  PS-Simulink Converter2/1 -> Display11/1, [io_source_3_3]
  [io_source_3_3] -> Add15/3
  [v_bus_3_3] -> Add16/3
  [io_source_1_3] -> Mux/1
  PS-Simulink Converter7/1 -> Display5/1
  PS-Simulink Converter4/1 -> [v_bus_1_3], Display1/1
  PS-Simulink Converter16/1 -> [i_cpl_3_3], Display3/1
  PS-Simulink Converter14/1 -> Display7/1, [i_cpl_2_3]
  [v_bus_2_3] -> Divide4/2
  [V_out1_3] -> Mux1/1
  Add15/1 -> To Workspace35/1, [i_MG_3]
  [V_out_source_1_3] -> Simulink-PS Converter/1
  Step17/1 -> Add46/2
  [v_bus_3_3] -> Divide5/2
  Gain5/1 -> [V_MG_3], To Workspace9/1
  [io_source_2_3] -> Add15/2
  [v_bus_1_3] -> Add16/1
  PS-Simulink Converter8/1 -> Display6/1
  Constant4/1 -> Add46/1
  PS-Simulink Converter13/1 -> [v_bus_2_3], Display8/1
  [V_out_source_3_3] -> Simulink-PS Converter11/1
  [io_source_3_3] -> Mux/3
  Divide5/1 -> Simulink-PS Converter1/1
  [io_source_1_3] -> Add15/1
  [V_out3_3] -> Mux1/3
  Add16/1 -> Gain5/1
  [v_bus_2_3] -> Add16/2
  [V_out_source_2_3] -> Simulink-PS Converter9/1
  [v_bus_1_3] -> Divide3/2
  PS-Simulink Converter/1 -> To Workspace/1, Display2/1, [io_source_1_3]
  Divide4/1 -> Simulink-PS Converter10/1
  Add46/1 -> Goto29/1
  PS-Simulink Converter5/1 -> [i_cpl_1_3], Display/1
  Divide3/1 -> Simulink-PS Converter8/1
  Mux/1 -> Scope/2
  PS-Simulink Converter15/1 -> [v_bus_3_3], Display10/1
  PS-Simulink Converter11/1 -> To Workspace1/1, Display9/1, [io_source_2_3]
  Mux1/1 -> Scope/1
  [V_out2_3] -> Mux1/2
  [io_source_2_3] -> Mux/2
  Sine Wave1/1 -> Add1/2
  Product1/1 -> ?
  Add1/1 -> Product1/1
  Constant1/1 -> Add1/1
  Step1/1 -> Product1/2
  Sum4/1 -> Scope2/1, Saturation5/1
  Sum12/1 -> Scope4/1, Saturation6/1
  Close loop equivalent1/1 -> [delta_V_3_3], Scope28/1
  Sum2/1 -> Scope3/1, Saturation4/1
  [V_ref_mg_3] -> Sum4/1
  [V_MG_3] -> [V_MG_tau_3]
  [V_MG_tau_3] -> Sum4/2
  [V_ref_mg_3] -> Sum2/1
  [V_MG_tau_3] -> Sum2/2
  [V_ref_mg_2] -> Sum12/1
  [V_MG_tau_3] -> Sum12/2
  Derivative/1 -> Scope1/1
  Add19/1 -> Scope6/1, Divide5/1
  Step2/1 -> Add2/1
  Add2/1 -> Scope7/1, Divide4/1
  Step4/1 -> Add2/2
  Step10/1 -> Add3/2
  Add3/1 -> Scope8/1, Divide3/1
  Step6/1 -> Add3/1
  Step3/1 -> Add2/3
  Step8/1 -> Add3/3
  Add4/1 -> Divide1/1, Scope15/1
  [V_MG_tau_3] -> Sum5/2
  [V_ref_mg_3] -> Sum5/1
  Close loop equivalent4/1 -> [delta_V_4_3], Scope12/1
  Sum5/1 -> Saturation1/1, Scope10/1
  PS-Simulink Converter9/1 -> Display12/1, [v_bus_4_3]
  PS-Simulink Converter18/1 -> Display4/1, [V_out4_3]
  Divide1/1 -> Simulink-PS Converter2/1
  [V_out_source_4_3] -> Simulink-PS Converter3/1
  [v_bus_4_3] -> Divide1/2
  PS-Simulink Converter10/1 -> Display14/1, [i_cpl_4_3]
  PS-Simulink Converter17/1 -> [io_source_4_3], Display13/1, To Workspace6/1
  From18/1 -> Close loop equivalent6/1
  Add7/1 -> [delta_I_4_3]
  [io_source_4_3] -> Gain2/1
  Gain1/1 -> Sum1/1, Sum3/1
  [V_REF_c] -> Add6/2
  [delta_I_4_3] -> Add6/1
  Gain2/1 -> Add7/2
  Add5/1 -> [V_out_source_4_3]
  [V_ref_tot_4_3] -> Add5/2
  Saturation1/1 -> Close loop equivalent4/1
  Integrator1/1 -> Sum3/2
  Manual Switch2/1 -> Add5/1
  [error_i_4_3] -> Integrator1/1
  [delta_V_4_3] -> Add6/3
  Constant2/1 -> Switch1/3
  Constant3/1 -> Manual Switch2/2
  Step11/1 -> Switch1/2
  Sum3/1 -> [i_prom_4_3], Scope14/1, Sum1/2
  [io_source_4_3] -> Gain1/1
  Switch1/1 -> Add7/1
  PI i1/1 -> Scope13/1, To Workspace7/1, Switch1/1
  Sum1/1 -> Saturation2/1
  Saturation2/1 -> Scope11/1, PI i1/1
  Add6/1 -> [V_ref_tot_4_3]
  Close loop equivalent6/1 -> Manual Switch2/1
  Step15/1 -> Add19/1
  Step18/1 -> Add19/2
  Step16/1 -> Add19/3
  Step5/1 -> Add4/1
  Step7/1 -> Add4/3
  Step9/1 -> Add4/2
  [v_bus_4_3] -> Add16/4
  [io_source_4_3] -> Add15/4
  [V_out4_3] -> Mux1/4
  [V_MG_3] -> Mux1/5
  [io_source_4_3] -> Mux/4
  [i_prom_4_3] -> Saturation3/1
  Saturation3/1 -> Mux7/4
  MATLAB Function1/4(error_4) -> [error_i_4_3]
  PS-Simulink Converter3/1 -> Display15/1, [V_out3_3]
  PS-Simulink Converter12/1 -> Display16/1, [V_out2_3]
  PS-Simulink Converter1/1 -> Display17/1, [V_out1_3]
  [V_ref_tot_1_3] -> Add33/2
  Constant5/1 -> MATLAB Function1/2(aij)
  Constant18/1 -> MATLAB Function2/2(aij)
  [V_ref_tot_1_4] -> Add17/2
  PS-Simulink Converter19/1 -> [V_out1_4], Display27/1
  PS-Simulink Converter22/1 -> [V_out2_4], Display26/1
  PS-Simulink Converter30/1 -> [V_out3_4], Display25/1
  MATLAB Function2/4(error_4) -> [error_i_4_4]
  Saturation19/1 -> Mux4/4
  [i_prom_4_4] -> Saturation19/1
  [io_source_4_4] -> Mux2/4
  [V_MG_4] -> Mux3/5
  [V_out4_4] -> Mux3/4
  [io_source_4_4] -> Add9/4
  [v_bus_4_4] -> Add10/4
  Step36/1 -> Add20/2
  Step33/1 -> Add20/3
  Step30/1 -> Add20/1
  Step20/1 -> Add11/3
  Step22/1 -> Add11/2
  Step19/1 -> Add11/1
  Close loop equivalent14/1 -> Manual Switch5/1
  Add29/1 -> [V_ref_tot_4_4]
  Saturation18/1 -> PI i2/1, Scope18/1
  Sum13/1 -> Saturation18/1
  PI i2/1 -> Switch2/1, To Workspace11/1, Scope20/1
  Switch2/1 -> Add30/1
  [io_source_4_4] -> Gain3/1
  Sum18/1 -> Sum13/2, Scope30/1, [i_prom_4_4]
  Step14/1 -> Switch2/2
  Constant16/1 -> Manual Switch5/2
  Constant10/1 -> Switch2/3
  [delta_V_4_4] -> Add29/3
  [error_i_4_4] -> Integrator2/1
  Manual Switch5/1 -> Add26/1
  Integrator2/1 -> Sum18/2
  Saturation7/1 -> Close loop equivalent13/1
  [V_ref_tot_4_4] -> Add26/2
  Add26/1 -> [V_out_source_4_4]
  Gain11/1 -> Add30/2
  [delta_I_4_4] -> Add29/1
  [V_REF_c] -> Add29/2
  Gain3/1 -> Sum18/1, Sum13/1
  [io_source_4_4] -> Gain11/1
  Add30/1 -> [delta_I_4_4]
  From77/1 -> Close loop equivalent14/1
  PS-Simulink Converter27/1 -> To Workspace10/1, Display23/1, [io_source_4_4]
  PS-Simulink Converter20/1 -> [i_cpl_4_4], Display24/1
  [v_bus_4_4] -> Divide2/2
  [V_out_source_4_4] -> Simulink-PS Converter13/1
  Divide2/1 -> Simulink-PS Converter12/1
  PS-Simulink Converter28/1 -> [V_out4_4], Display30/1
  PS-Simulink Converter35/1 -> [v_bus_4_4], Display22/1
  Sum20/1 -> Scope17/1, Saturation7/1
  Close loop equivalent13/1 -> Scope19/1, [delta_V_4_4]
  [V_ref_mg_4] -> Sum20/1
  [V_MG_tau_4] -> Sum20/2
  Add20/1 -> Scope31/1, Divide2/1
  Step34/1 -> Add13/3
  Step25/1 -> Add12/3
  Step31/1 -> Add13/1
  Add13/1 -> Divide6/1, Scope47/1
  Step13/1 -> Add13/2
  Step29/1 -> Add12/2
  Add12/1 -> Divide7/1, Scope46/1
  Step23/1 -> Add12/1
  Add11/1 -> Divide8/1, Scope45/1
  Derivative1/1 -> Scope16/1
  [V_MG_tau_4] -> Sum16/2
  [V_ref_mg_4] -> Sum16/1
  [V_MG_tau_4] -> Sum17/2
  [V_ref_mg_4] -> Sum17/1
  [V_MG_tau_4] -> Sum19/2
  [V_MG_4] -> [V_MG_tau_4]
  [V_ref_mg_4] -> Sum19/1
  Sum17/1 -> Saturation20/1, Scope42/1
  Close loop equivalent5/1 -> Scope40/1, [delta_V_3_4]
  Sum16/1 -> Saturation22/1, Scope43/1
  Sum19/1 -> Saturation21/1, Scope32/1
  Step12/1 -> Product2/2
  Constant6/1 -> Add8/1
  Add8/1 -> Product2/1
  Product2/1 -> ?
  Sine Wave2/1 -> Add8/2
  [io_source_2_4] -> Mux2/2
  [V_out2_4] -> Mux3/2
  Mux3/1 -> Scope9/1
  PS-Simulink Converter21/1 -> [io_source_2_4], Display35/1, To Workspace3/1
  PS-Simulink Converter25/1 -> Display20/1, [v_bus_3_4]
  Mux2/1 -> Scope9/2
  Divide6/1 -> Simulink-PS Converter14/1
  PS-Simulink Converter32/1 -> Display18/1, [i_cpl_1_4]
  Add24/1 -> Goto44/1
  Divide7/1 -> Simulink-PS Converter6/1
  PS-Simulink Converter6/1 -> [io_source_1_4], Display28/1, To Workspace2/1
  [v_bus_1_4] -> Divide6/2
  [V_out_source_2_4] -> Simulink-PS Converter15/1
  [v_bus_2_4] -> Add10/2
  Add10/1 -> Gain14/1
  [V_out3_4] -> Mux3/3
  [io_source_1_4] -> Add9/1
  Divide8/1 -> Simulink-PS Converter5/1
  [io_source_3_4] -> Mux2/3
  [V_out_source_3_4] -> Simulink-PS Converter7/1
  PS-Simulink Converter23/1 -> Display34/1, [v_bus_2_4]
  Constant17/1 -> Add24/1
  PS-Simulink Converter34/1 -> Display32/1
  [v_bus_1_4] -> Add10/1
  [io_source_2_4] -> Add9/2
  Gain14/1 -> To Workspace12/1, [V_MG_4]
  [v_bus_3_4] -> Divide8/2
  Step21/1 -> Add24/2
  [V_out_source_1_4] -> Simulink-PS Converter4/1
  Add9/1 -> To Workspace34/1, [i_MG_4]
  [V_out1_4] -> Mux3/1
  [v_bus_2_4] -> Divide7/2
  PS-Simulink Converter24/1 -> [i_cpl_2_4], Display33/1
  PS-Simulink Converter26/1 -> Display29/1, [i_cpl_3_4]
  PS-Simulink Converter31/1 -> Display19/1, [v_bus_1_4]
  PS-Simulink Converter33/1 -> Display31/1
  [io_source_1_4] -> Mux2/1
  [v_bus_3_4] -> Add10/3
  [io_source_3_4] -> Add9/3
  PS-Simulink Converter29/1 -> [io_source_3_4], Display21/1
  From56/1 -> Close loop equivalent11/1
  Add22/1 -> [V_ref_tot_1_4]
  [delta_I_2_4] -> Add27/1
  [io_source_1_4] -> Gain9/1
  PI i 1/1 -> Switch4/1, Scope36/1, To Workspace5/1
  Gain10/1 -> Add23/2
  Gain9/1 -> Sum23/1, Sum24/1
  Close loop equivalent12/1 -> [delta_V_1_4], Scope37/1
  [io_source_2_4] -> Gain4/1
  Add21/1 -> [delta_I_3_4]
  Constant9/1 -> Manual Switch1/2
  Step26/1 -> Switch3/2
  [error_i_2_4] -> Integrator6/1
  [io_source_3_4] -> Gain8/1
  Integrator6/1 -> Sum22/2
  Mux4/1 -> MATLAB Function2/1(i)
  Close loop equivalent8/1 -> [delta_V_2_4], Scope38/1
  Add17/1 -> [V_out_source_1_4]
  [delta_I_1_4] -> Add22/1
  Gain6/1 -> Sum14/1, Sum15/1
  Add27/1 -> [V_ref_tot_2_4]
  Switch3/1 -> Add23/1
  [V_REF_c] -> Add18/2
  From54/1 -> Close loop equivalent10/1
  [delta_I_3_4] -> Add18/1
  PI i3/1 -> Switch3/1, Scope34/1, To Workspace4/1
  Gain8/1 -> Add21/2
  From47/1 -> Close loop equivalent9/1
  Add14/1 -> [V_out_source_3_4]
  Close loop equivalent9/1 -> Manual Switch4/1
  MATLAB Function2/1(error_1) -> [error_i_1_4]
  [i_prom_3_4] -> Saturation15/1
  Close loop equivalent10/1 -> Manual Switch1/1
  Integrator7/1 -> Sum24/2
  Gain4/1 -> Sum22/1, Sum21/1
  Sum23/1 -> Saturation24/1
  Sum22/1 -> Sum21/2, [i_prom_2_4]
  Saturation22/1 -> Close loop equivalent12/1
  MATLAB Function2/2(error_2) -> [error_i_2_4]
  [delta_V_1_4] -> Add22/3
  Saturation24/1 -> Scope33/1, PI i3/1
  [V_ref_tot_3_4] -> Add14/2
  Saturation20/1 -> Close loop equivalent8/1
  Saturation21/1 -> Close loop equivalent5/1
  Saturation15/1 -> Mux4/3
  [io_source_1_4] -> Gain10/1
  Integrator8/1 -> Sum15/2
  Saturation14/1 -> Scope35/1, PI i 1/1
  [V_REF_c] -> Add27/2
  Manual Switch3/1 -> Add14/1
  [error_i_3_4] -> Integrator8/1
  [delta_V_3_4] -> Add18/3
  Constant11/1 -> Switch5/3
  Constant12/1 -> Manual Switch3/2
  Step24/1 -> Switch5/2
  [i_prom_2_4] -> Saturation16/1
  Sum21/1 -> Saturation14/1
  [error_i_1_4] -> Integrator7/1
  Add23/1 -> [delta_I_1_4]
  Add25/1 -> [V_out_source_2_4]
  [io_source_2_4] -> Gain7/1
  Sum15/1 -> [i_prom_3_4], Scope44/1, Sum14/2
  [io_source_3_4] -> Gain6/1
  Switch5/1 -> Add21/1
  [i_prom_1_4] -> Saturation17/1
  Manual Switch1/1 -> Add17/1
  PI i6/1 -> Scope41/1, To Workspace8/1, Switch5/1
  Step27/1 -> Switch4/2
  Saturation17/1 -> Mux4/1
  Saturation16/1 -> Mux4/2
  Sum14/1 -> Saturation23/1
  Saturation23/1 -> Scope39/1, PI i6/1
  Sum24/1 -> [i_prom_1_4], Sum23/2
  Manual Switch4/1 -> Add25/1
  Constant7/1 -> Switch4/3
  Add18/1 -> [V_ref_tot_3_4]
  [V_ref_tot_2_4] -> Add25/2
  Constant15/1 -> Manual Switch4/2
  [delta_V_2_4] -> Add27/3
  Close loop equivalent11/1 -> Manual Switch3/1
  Switch4/1 -> Add28/1
  Gain7/1 -> Add28/2
  Add28/1 -> [delta_I_2_4]
  [V_REF_c] -> Add22/2
  MATLAB Function2/3(error_3) -> [error_i_3_4]
  Constant8/1 -> Switch3/3
  Constant33/1 -> MATLAB Function3/2(aij)
  [V_ref_tot_1_1] -> Add41/2
  PS-Simulink Converter37/1 -> [V_out1_1], Display45/1
  PS-Simulink Converter40/1 -> [V_out2_1], Display44/1
  PS-Simulink Converter48/1 -> [V_out3_1], Display43/1
  Step41/1 -> Add36/3
  Step43/1 -> Add36/2
  Step40/1 -> Add36/1
  Step53/1 -> Add38/3
  Step46/1 -> Add37/3
  Step51/1 -> Add38/1
  Add38/1 -> Divide10/1, Scope71/1
  Step38/1 -> Add38/2
  Step49/1 -> Add37/2
  Add37/1 -> Divide11/1, Scope70/1
  Step44/1 -> Add37/1
  Add36/1 -> Divide12/1, Scope69/1
  [V_MG_tau_1] -> Sum28/2
  [V_ref_mg_1] -> Sum28/1
  [V_MG_tau_1] -> Sum29/2
  [V_ref_mg_1] -> Sum29/1
  [V_MG_tau_1] -> Sum31/2
  [V_MG_1] -> [V_MG_tau_1]
  [V_ref_mg_1] -> Sum31/1
  Sum29/1 -> Saturation32/1, Scope66/1
  Close loop equivalent15/1 -> Scope64/1, [delta_V_3_1]
  Sum28/1 -> Saturation34/1, Scope67/1
  Sum31/1 -> Saturation33/1, Scope56/1
  Step37/1 -> Product3/2
  Constant23/1 -> Add32/1
  Add32/1 -> Product3/1
  Product3/1 -> ?
  Sine Wave3/1 -> Add32/2
  [io_source_2_1] -> Mux5/2
  [V_out2_1] -> Mux6/2
  Mux6/1 -> Scope48/1
  PS-Simulink Converter39/1 -> [io_source_2_1], Display53/1, To Workspace14/1
  PS-Simulink Converter43/1 -> Display38/1, [v_bus_3_1]
  Mux5/1 -> Scope48/2
  Divide10/1 -> Simulink-PS Converter22/1
  PS-Simulink Converter50/1 -> Display36/1, [i_cpl_1_1]
  Add54/1 -> Goto106/1
  Divide11/1 -> Simulink-PS Converter18/1
  PS-Simulink Converter36/1 -> [io_source_1_1], Display46/1, To Workspace13/1
  [v_bus_1_1] -> Divide10/2
  [V_out_source_2_1] -> Simulink-PS Converter23/1
  [v_bus_2_1] -> Add35/2
  Add35/1 -> Gain27/1
  [V_out3_1] -> Mux6/3
  [io_source_1_1] -> Add34/1
  Divide12/1 -> Simulink-PS Converter17/1
  [io_source_3_1] -> Mux5/3
  [V_out_source_3_1] -> Simulink-PS Converter19/1
  PS-Simulink Converter41/1 -> Display52/1, [v_bus_2_1]
  Constant32/1 -> Add54/1
  PS-Simulink Converter52/1 -> Display50/1
  [v_bus_1_1] -> Add35/1
  [io_source_2_1] -> Add34/2
  Gain27/1 -> To Workspace23/1, [V_MG_1]
  [v_bus_3_1] -> Divide12/2
  Step42/1 -> Add54/2
  [V_out_source_1_1] -> Simulink-PS Converter16/1
  Add34/1 -> To Workspace33/1, [i_MG_1]
  [V_out1_1] -> Mux6/1
  [v_bus_2_1] -> Divide11/2
  PS-Simulink Converter42/1 -> [i_cpl_2_1], Display51/1
  PS-Simulink Converter44/1 -> Display47/1, [i_cpl_3_1]
  PS-Simulink Converter49/1 -> Display37/1, [v_bus_1_1]
  PS-Simulink Converter51/1 -> Display49/1
  [io_source_1_1] -> Mux5/1
  [v_bus_3_1] -> Add35/3
  [io_source_3_1] -> Add34/3
  PS-Simulink Converter47/1 -> [io_source_3_1], Display39/1
  From153/1 -> Close loop equivalent21/1
  Add52/1 -> [V_ref_tot_1_1]
  [delta_I_2_1] -> Add57/1
  [io_source_1_1] -> Gain24/1
  PI i 2/1 -> Switch8/1, Scope60/1, To Workspace16/1
  Gain25/1 -> Add53/2
  Gain24/1 -> Sum35/1, Sum36/1
  Close loop equivalent24/1 -> [delta_V_1_1], Scope61/1
  [io_source_2_1] -> Gain20/1
  Add48/1 -> [delta_I_3_1]
  Constant26/1 -> Manual Switch6/2
  Step47/1 -> Switch7/2
  [error_i_2_1] -> Integrator10/1
  [io_source_3_1] -> Gain23/1
  Integrator10/1 -> Sum34/2
  Mux8/1 -> MATLAB Function3/1(i)
  Close loop equivalent17/1 -> [delta_V_2_1], Scope62/1
  Add41/1 -> [V_out_source_1_1]
  [delta_I_1_1] -> Add52/1
  Gain21/1 -> Sum26/1, Sum27/1
  Add57/1 -> [V_ref_tot_2_1]
  Switch7/1 -> Add53/1
  [V_REF_c] -> Add43/2
  From151/1 -> Close loop equivalent20/1
  [delta_I_3_1] -> Add43/1
  PI i8/1 -> Switch7/1, Scope58/1, To Workspace15/1
  Gain23/1 -> Add48/2
  From144/1 -> Close loop equivalent18/1
  Add40/1 -> [V_out_source_3_1]
  Close loop equivalent18/1 -> Manual Switch8/1
  MATLAB Function3/1(error_1) -> [error_i_1_1]
  [i_prom_3_1] -> Saturation27/1
  Close loop equivalent20/1 -> Manual Switch6/1
  Integrator11/1 -> Sum36/2
  Gain20/1 -> Sum34/1, Sum33/1
  Sum35/1 -> Saturation36/1
  Sum34/1 -> Sum33/2, [i_prom_2_1]
  Saturation34/1 -> Close loop equivalent24/1
  MATLAB Function3/2(error_2) -> [error_i_2_1]
  [delta_V_1_1] -> Add52/3
  Saturation36/1 -> Scope57/1, PI i8/1
  [V_ref_tot_3_1] -> Add40/2
  Saturation32/1 -> Close loop equivalent17/1
  Saturation33/1 -> Close loop equivalent15/1
  Saturation27/1 -> Mux8/3
  [io_source_1_1] -> Gain25/1
  Integrator12/1 -> Sum27/2
  Saturation26/1 -> Scope59/1, PI i 2/1
  [V_REF_c] -> Add57/2
  Manual Switch7/1 -> Add40/1
  [error_i_3_1] -> Integrator12/1
  [delta_V_3_1] -> Add43/3
  Constant28/1 -> Switch9/3
  Constant29/1 -> Manual Switch7/2
  Step45/1 -> Switch9/2
  [i_prom_2_1] -> Saturation28/1
  Sum33/1 -> Saturation26/1
  [error_i_1_1] -> Integrator11/1
  Add53/1 -> [delta_I_1_1]
  Add55/1 -> [V_out_source_2_1]
  [io_source_2_1] -> Gain22/1
  Sum27/1 -> [i_prom_3_1], Scope68/1, Sum26/2
  [io_source_3_1] -> Gain21/1
  Switch9/1 -> Add48/1
  [i_prom_1_1] -> Saturation29/1
  Manual Switch6/1 -> Add41/1
  PI i9/1 -> Scope65/1, To Workspace17/1, Switch9/1
  Step48/1 -> Switch8/2
  Saturation29/1 -> Mux8/1
  Saturation28/1 -> Mux8/2
  Sum26/1 -> Saturation35/1
  Saturation35/1 -> Scope63/1, PI i9/1
  Sum36/1 -> [i_prom_1_1], Sum35/2
  Manual Switch8/1 -> Add55/1
  Constant24/1 -> Switch8/3
  Add43/1 -> [V_ref_tot_3_1]
  [V_ref_tot_2_1] -> Add55/2
  Constant30/1 -> Manual Switch8/2
  [delta_V_2_1] -> Add57/3
  Close loop equivalent21/1 -> Manual Switch7/1
  Switch8/1 -> Add58/1
  Gain22/1 -> Add58/2
  Add58/1 -> [delta_I_2_1]
  [V_REF_c] -> Add52/2
  MATLAB Function3/3(error_3) -> [error_i_3_1]
  Constant25/1 -> Switch7/3
  [V_MG_1] -> Mux6/4
  [V_MG_2] -> Mux10/3
  Constant34/1 -> Switch6/3
  [V_REF_c] -> Add67/2
  Add72/1 -> [delta_I_2_2]
  Gain28/1 -> Add72/2
  Switch10/1 -> Add72/1
  [delta_V_2_2] -> Add71/3
  Constant38/1 -> Manual Switch11/2
  [V_ref_tot_2_2] -> Add70/2
  Constant31/1 -> Switch10/3
  Manual Switch11/1 -> Add70/1
  Sum42/1 -> Sum41/2, [i_prom_1_2]
  Saturation31/1 -> Mux11/2
  Saturation37/1 -> Mux11/1
  Step61/1 -> Switch10/2
  Manual Switch9/1 -> Add64/1
  [i_prom_1_2] -> Saturation37/1
  [io_source_2_2] -> Gain28/1
  Add70/1 -> [V_out_source_2_2]
  Add68/1 -> [delta_I_1_2]
  [error_i_1_2] -> Integrator13/1
  Sum39/1 -> Saturation25/1
  [i_prom_2_2] -> Saturation31/1
  [V_REF_c] -> Add71/2
  Saturation25/1 -> PI i 4/1, Scope53/1
  [io_source_1_2] -> Gain31/1
  Saturation38/1 -> Close loop equivalent28/1
  Saturation42/1 -> PI i7/1, Scope51/1
  [delta_V_1_2] -> Add67/3
  MATLAB Function4/2(error_2) -> [error_i_2_2]
  Saturation40/1 -> Close loop equivalent32/1
  Sum40/1 -> [i_prom_2_2], Sum39/2
  Sum41/1 -> Saturation42/1
  Gain19/1 -> Sum39/1, Sum40/1
  Integrator13/1 -> Sum42/2
  Close loop equivalent30/1 -> Manual Switch9/1
  MATLAB Function4/1(error_1) -> [error_i_1_2]
  Close loop equivalent29/1 -> Manual Switch11/1
  From172/1 -> Close loop equivalent29/1
  PI i7/1 -> To Workspace24/1, Scope52/1, Switch6/1
  From182/1 -> Close loop equivalent30/1
  Switch6/1 -> Add68/1
  Add71/1 -> [V_ref_tot_2_2]
  [delta_I_1_2] -> Add67/1
  Add64/1 -> [V_out_source_1_2]
  Close loop equivalent28/1 -> [delta_V_2_2], Scope72/1
  Mux11/1 -> MATLAB Function4/1(i)
  Integrator9/1 -> Sum40/2
  [error_i_2_2] -> Integrator9/1
  Step60/1 -> Switch6/2
  Constant35/1 -> Manual Switch9/2
  [io_source_2_2] -> Gain19/1
  Close loop equivalent32/1 -> Scope55/1, [delta_V_1_2]
  Gain30/1 -> Sum42/1, Sum41/1
  Gain31/1 -> Add68/2
  PI i 4/1 -> To Workspace25/1, Scope54/1, Switch10/1
  [io_source_1_2] -> Gain30/1
  [delta_I_2_2] -> Add71/1
  Add67/1 -> [V_ref_tot_1_2]
  [io_source_1_2] -> Mux9/1
  PS-Simulink Converter62/1 -> Display59/1
  PS-Simulink Converter60/1 -> [v_bus_1_2], Display41/1
  PS-Simulink Converter55/1 -> Display61/1, [i_cpl_2_2]
  [v_bus_2_2] -> Divide13/2
  [V_out1_2] -> Mux10/1
  Add56/1 -> To Workspace32/1, [i_MG_2]
  [V_out_source_1_2] -> Simulink-PS Converter20/1
  Step55/1 -> Add69/2
  Gain32/1 -> [V_MG_2], To Workspace27/1
  [io_source_2_2] -> Add56/2
  [v_bus_1_2] -> Add59/1
  Constant39/1 -> Add69/1
  PS-Simulink Converter54/1 -> [v_bus_2_2], Display62/1
  [io_source_1_2] -> Add56/1
  Add59/1 -> Gain32/1
  [v_bus_2_2] -> Add59/2
  [V_out_source_2_2] -> Simulink-PS Converter27/1
  [v_bus_1_2] -> Divide9/2
  PS-Simulink Converter38/1 -> To Workspace18/1, Display57/1, [io_source_1_2]
  Divide13/1 -> Simulink-PS Converter24/1
  Add69/1 -> Goto94/1
  PS-Simulink Converter61/1 -> [i_cpl_1_2], Display40/1
  Divide9/1 -> Simulink-PS Converter26/1
  Mux9/1 -> Scope49/2
  PS-Simulink Converter46/1 -> To Workspace19/1, Display63/1, [io_source_2_2]
  Mux10/1 -> Scope49/1
  [V_out2_2] -> Mux10/2
  [io_source_2_2] -> Mux9/2
  Sine Wave4/1 -> Add47/2
  Add47/1 -> Product4/1
  Constant27/1 -> Add47/1
  Step39/1 -> Product4/2
  Sum32/1 -> Scope77/1, Saturation40/1
  Sum37/1 -> Scope76/1, Saturation38/1
  [V_MG_2] -> [V_MG_tau_2]
  [V_ref_mg_2] -> Sum37/1
  [V_MG_tau_2] -> Sum37/2
  [V_ref_mg_2] -> Sum32/1
  [V_MG_tau_2] -> Sum32/2
  Step57/1 -> Add61/1
  Add61/1 -> Scope80/1, Divide13/1
  Step62/1 -> Add61/2
  Step50/1 -> Add62/2
  Add62/1 -> Scope81/1, Divide9/1
  Step63/1 -> Add62/1
  Step59/1 -> Add61/3
  Step64/1 -> Add62/3
  PS-Simulink Converter53/1 -> Display55/1, [V_out2_2]
  PS-Simulink Converter45/1 -> Display56/1, [V_out1_2]
  [V_ref_tot_1_2] -> Add64/2
  Constant40/1 -> MATLAB Function4/2(aij)
  Constant36/1 -> Switch11/3
  [V_REF_c] -> Add63/2
  Sum38/1 -> Sum30/2, [i_prom_1]
  Manual Switch10/1 -> Add60/1
  Switch11/1 -> [delta_I_1]
  [error_i_1] -> Integrator14/1
  [delta_V_1] -> Add63/3
  Saturation30/1 -> Close loop equivalent33/1
  Sum30/1 -> Saturation39/1
  Integrator14/1 -> Sum38/2
  Close loop equivalent31/1 -> Manual Switch10/1
  From161/1 -> Close loop equivalent31/1
  [delta_I_1] -> Add63/1
  Add60/1 -> [V_ref_mg_1]
  Step52/1 -> Switch11/2
  Constant37/1 -> Manual Switch10/2
  Close loop equivalent33/1 -> Scope74/1, [delta_V_1]
  Gain26/1 -> Sum38/1, Sum30/1
  [i_MG_1] -> Gain26/1
  Add63/1 -> [V_ref_tot_1]
  Sum25/1 -> Scope75/1, Saturation30/1
  [V_REF_c] -> Sum25/1
  [V_MG_tau] -> Sum25/2
  [V_ref_tot_1] -> Add60/2
  MATLAB Function5/3(error_3) -> [error_i_3]
  Saturation43/1 -> Mux12/2
  Saturation44/1 -> Mux12/1
  [i_prom_1] -> Saturation44/1
  [i_prom_2] -> Saturation43/1
  Saturation41/1 -> Mux12/3
  MATLAB Function5/2(error_2) -> [error_i_2]
  [i_prom_3] -> Saturation41/1
  MATLAB Function5/1(error_1) -> [error_i_1]
  Sine Wave5/1 -> Add66/2
  Product5/1 -> Scope95/1, Variable Time Delay/2
  Add66/1 -> Product5/1
  Constant41/1 -> Add66/1
  [V_MG_3] -> Add73/3
  Step56/1 -> Add74/2
  Gain33/1 -> [V_MG], To Workspace28/1
  [V_MG_1] -> Add73/1
  Constant43/1 -> Add74/1
  Add73/1 -> Gain33/1
  [V_MG_2] -> Add73/2
  Add74/1 -> [V_REF_c]
  [V_ref_tot_2] -> Add65/2
  [V_MG_tau] -> Sum43/2
  [V_REF_c] -> Sum43/1
  Sum43/1 -> Saturation45/1, Scope83/1
  Add75/1 -> [V_ref_tot_2]
  [i_MG_2] -> Gain29/1
  Gain29/1 -> Sum44/1, Sum45/1
  Close loop equivalent36/1 -> [delta_V_2], Scope82/1
  Constant45/1 -> Manual Switch12/2
  Step58/1 -> Switch12/2
  Add65/1 -> [V_ref_mg_2]
  [delta_I_2] -> Add75/1
  From247/1 -> Close loop equivalent35/1
  Subsystem/1(Out1) -> Switch12/1, Scope79/1, To Workspace29/1
  Close loop equivalent35/1 -> Manual Switch12/1
  Integrator15/1 -> Sum45/2
  Sum44/1 -> Saturation46/1
  Saturation45/1 -> Close loop equivalent36/1
  [delta_V_2] -> Add75/3
  Saturation46/1 -> Subsystem/2(In2), Subsystem/1(In1), Scope78/1
  [error_i_2] -> Integrator15/1
  Switch12/1 -> [delta_I_2]
  Manual Switch12/1 -> Add65/1
  Sum45/1 -> [i_prom_2], Sum44/2
  [V_REF_c] -> Add75/2
  Constant44/1 -> Switch12/3
  Constant46/1 -> Switch13/3
  [V_REF_c] -> Add77/2
  Sum48/1 -> Sum47/2, [i_prom_3]
  Manual Switch14/1 -> Add76/1
  Switch13/1 -> [delta_I_3]
  [error_i_3] -> Integrator16/1
  Saturation48/1 -> Subsystem2/1(In1), Subsystem2/2(In2), Scope84/1
  [delta_V_3] -> Add77/3
  Saturation47/1 -> Close loop equivalent39/1
  Sum47/1 -> Saturation48/1
  Integrator16/1 -> Sum48/2
  Close loop equivalent38/1 -> Manual Switch14/1
  Subsystem2/1(Out1) -> To Workspace30/1, Scope85/1, Switch13/1
  From256/1 -> Close loop equivalent38/1
  [delta_I_3] -> Add77/1
  Add76/1 -> [V_ref_mg_3]
  Step65/1 -> Switch13/2
  Constant47/1 -> Manual Switch14/2
  Close loop equivalent39/1 -> Scope86/1, [delta_V_3]
  Gain34/1 -> Sum48/1, Sum47/1
  [i_MG_3] -> Gain34/1
  Add77/1 -> [V_ref_tot_3]
  Sum46/1 -> Scope87/1, Saturation47/1
  [V_REF_c] -> Sum46/1
  [V_MG_tau] -> Sum46/2
  [V_ref_tot_3] -> Add76/2
  [V_ref_tot_4] -> Add78/2
  [V_MG_tau] -> Sum49/2
  [V_REF_c] -> Sum49/1
  Sum49/1 -> Saturation49/1, Scope91/1
  Add79/1 -> [V_ref_tot_4]
  [i_MG_4] -> Gain35/1
  Gain35/1 -> Sum50/1, Sum51/1
  Close loop equivalent42/1 -> [delta_V_4], Scope90/1
  Constant49/1 -> Manual Switch15/2
  Step66/1 -> Switch14/2
  Add78/1 -> [V_ref_mg_4]
  [delta_I_4] -> Add79/1
  From265/1 -> Close loop equivalent41/1
  Subsystem3/1(Out1) -> Switch14/1, Scope89/1, To Workspace31/1
  Close loop equivalent41/1 -> Manual Switch15/1
  Integrator17/1 -> Sum51/2
  Sum50/1 -> Saturation50/1
  Saturation49/1 -> Close loop equivalent42/1
  [delta_V_4] -> Add79/3
  Saturation50/1 -> Subsystem3/1(In1), Subsystem3/2(In2), Scope88/1
  [error_i_4] -> Integrator17/1
  Switch14/1 -> [delta_I_4]
  Manual Switch15/1 -> Add78/1
  Sum51/1 -> [i_prom_4], Sum50/2
  [V_REF_c] -> Add79/2
  Constant48/1 -> Switch14/3
  [i_prom_4] -> Saturation51/1
  Saturation51/1 -> Mux12/4
  MATLAB Function5/4(error_4) -> [error_i_4]
  [V_MG_4] -> Add73/4
  [i_MG_1] -> Mux13/1
  [V_MG_3] -> Mux14/3
  [V_MG_1] -> Mux14/1
  [i_MG_2] -> Mux13/2
  Mux14/1 -> Scope92/1
  [i_MG_3] -> Mux13/3
  [i_MG_4] -> Mux13/4
  [V_MG_2] -> Mux14/2
  [V_MG_4] -> Mux14/4
  Mux13/1 -> Scope92/2
  [V_MG] -> Mux14/5
  [V_MG] -> Variable Time Delay/1
  Variable Time Delay/1 -> [V_MG_tau]
  Add80/1 -> Scope93/1, Product6/1
  Sine Wave6/1 -> Add80/2
  Mux12/1 -> Variable Time Delay1/1
  Variable Time Delay1/1 -> MATLAB Function5/1(i)
  Constant50/1 -> Add80/1
  Step68/1 -> Add81/2
  Constant42/1 -> Add81/1
  Add81/1 -> MATLAB Function5/2(aij)
  Step69/1 -> Add81/3
  Step54/1 -> Add82/1
  Add82/1 -> Product5/2
  Step70/1 -> Add82/2
  Step72/1 -> Add83/2
  Add83/1 -> Product6/2
  Step71/1 -> Add83/1
  Step67/1 -> Add38/4
  Step73/1 -> Add37/4
  Step74/1 -> Add36/4
  Step75/1 -> Add62/4
  Step76/1 -> Add61/4
  Step77/1 -> Add3/4
  Step79/1 -> Add4/4
  Step80/1 -> Add19/4
  Step78/1 -> Add2/4
  Step81/1 -> Add20/4
  Step82/1 -> Add11/4
  Step83/1 -> Add12/4
  Step84/1 -> Add13/4
  Saturation39/1 -> Subsystem1/2(In2), Subsystem1/1(In1), Scope50/1
  Subsystem1/1(Out1) -> Switch11/1
  Product6/1 -> Scope94/1, Variable Time Delay1/2
  Step85/1 -> Add82/3
  Step86/1 -> Add83/3
  connections:
  Voltage output 2/RConn2 -- Controlled Voltage Source3/RConn2 -- Electrical Reference1/LConn1 -- C bus 2/RConn1 -- Voltage bus 2/RConn2 -- Controlled Current Source6/LConn1
  Controlled Voltage Source1/RConn2 -- Controlled Current Source7/LConn1 -- Voltage bus 3/RConn2 -- C bus 3/RConn1 -- Voltage output 3/RConn2 -- Electrical Reference2/LConn1
  Current output 3/LConn1 -- Voltage output 3/LConn1 -- Controlled Voltage Source1/LConn1
  Voltage bus 1/LConn1 -- R serie 30/LConn1 -- R serie 18/RConn1 -- Current output 6/LConn1 -- Current load 1/LConn1 -- Current output 4/LConn1 -- C bus 1/LConn1 -- L serie 1/RConn1
  Voltage bus 4/LConn1 -- Current load 4/LConn1 -- R serie 5/RConn1 -- R serie 6/RConn1 -- C bus 4/LConn1 -- L serie 4/RConn1
  Current output 2/LConn1 -- Controlled Voltage Source3/LConn1 -- Voltage output 2/LConn1
  C bus 1/RConn1 -- Voltage bus 1/RConn2 -- Controlled Current Source5/LConn1 -- Controlled Voltage Source/RConn2 -- Solver Configuration/RConn1 -- Voltage output 1/RConn2 -- Electrical Reference/LConn1
  Voltage output 1/LConn1 -- Controlled Voltage Source/LConn1 -- Current output 1/LConn1
  L serie 2/LConn1 -- R serie 2/RConn1
  PS-Simulink Converter15/LConn1 -- Voltage bus 3/RConn1
  Current output 6/RConn1 -- PS-Simulink Converter8/LConn1
  PS-Simulink Converter1/LConn1 -- Voltage output 1/RConn1
  Current load 1/RConn1 -- PS-Simulink Converter5/LConn1
  PS-Simulink Converter13/LConn1 -- Voltage bus 2/RConn1
  Controlled Current Source7/RConn2 -- Current load 3/RConn2
  R serie 3/LConn1 -- Current output 3/RConn2
  Current output 6/RConn2 -- R serie 13/LConn1
  Controlled Current Source5/RConn2 -- Current load 1/RConn2
  PS-Simulink Converter2/LConn1 -- Current output 3/RConn1
  PS-Simulink Converter3/LConn1 -- Voltage output 3/RConn1
  PS-Simulink Converter4/LConn1 -- Voltage bus 1/RConn1
  Simulink-PS Converter11/RConn1 -- Controlled Voltage Source1/RConn1
  Current output 4/RConn2 -- R serie 12/LConn1
  L serie 3/LConn1 -- R serie 3/RConn1
  PS-Simulink Converter/LConn1 -- Current output 1/RConn1
  Simulink-PS Converter1/RConn1 -- Controlled Current Source7/RConn1
  Simulink-PS Converter9/RConn1 -- Controlled Voltage Source3/RConn1
  Current load 3/RConn1 -- PS-Simulink Converter16/LConn1
  PS-Simulink Converter12/LConn1 -- Voltage output 2/RConn1
  PS-Simulink Converter7/LConn1 -- Current output 4/RConn1
  Current load 2/RConn1 -- PS-Simulink Converter14/LConn1
  Controlled Current Source6/RConn2 -- Current load 2/RConn2
  Simulink-PS Converter8/RConn1 -- Controlled Current Source5/RConn1
  PS-Simulink Converter11/LConn1 -- Current output 2/RConn1
  L serie 1/LConn1 -- R serie 1/RConn1
  Simulink-PS Converter/RConn1 -- Controlled Voltage Source/RConn1
  Simulink-PS Converter10/RConn1 -- Controlled Current Source6/RConn1
  R serie 1/LConn1 -- Current output 1/RConn2
  R serie 2/LConn1 -- Current output 2/RConn2
  Controlled Voltage Source2/RConn2 -- Electrical Reference3/LConn1 -- Voltage output 4/RConn2 -- C bus 4/RConn1 -- Voltage bus 4/RConn2 -- Controlled Current Source1/LConn1
  Current output 7/LConn1 -- Controlled Voltage Source2/LConn1 -- Voltage output 4/LConn1
  Current load 4/RConn1 -- PS-Simulink Converter10/LConn1
  L serie 4/LConn1 -- R serie 4/RConn1
  Simulink-PS Converter2/RConn1 -- Controlled Current Source1/RConn1
  Simulink-PS Converter3/RConn1 -- Controlled Voltage Source2/RConn1
  Controlled Current Source1/RConn2 -- Current load 4/RConn2
  R serie 4/LConn1 -- Current output 7/RConn2
  PS-Simulink Converter9/LConn1 -- Voltage bus 4/RConn1
  PS-Simulink Converter18/LConn1 -- Voltage output 4/RConn1
  PS-Simulink Converter17/LConn1 -- Current output 7/RConn1
  R serie 12/RConn1 -- Current load 2/LConn1 -- R serie 5/LConn1 -- Voltage bus 2/LConn1 -- C bus 2/LConn1 -- L serie 2/RConn1
  R serie 6/LConn1 -- R serie 13/RConn1 -- Current load 3/LConn1 -- Voltage bus 3/LConn1 -- C bus 3/LConn1 -- L serie 3/RConn1
  Voltage output 6/RConn2 -- Controlled Current Source4/LConn1 -- Voltage bus 6/RConn2 -- C bus 6/RConn1 -- Electrical Reference5/LConn1 -- Controlled Voltage Source7/RConn2
  Controlled Voltage Source5/RConn2 -- Electrical Reference6/LConn1 -- Voltage output 7/RConn2 -- C bus 7/RConn1 -- Voltage bus 7/RConn2 -- Controlled Current Source8/LConn1
  Current output 9/LConn1 -- Controlled Voltage Source5/LConn1 -- Voltage output 7/LConn1
  Voltage bus 5/LConn1 -- R serie 18/LConn1 -- Current output 10/LConn1 -- R serie 29/LConn1 -- Current load 5/LConn1 -- Current output 11/LConn1 -- L serie 5/RConn1 -- C bus 5/LConn1
  Voltage bus 8/LConn1 -- R serie 15/RConn1 -- Current load 8/LConn1 -- R serie 16/RConn1 -- L serie 8/RConn1 -- C bus 8/LConn1
  Current output 8/LConn1 -- Voltage output 6/LConn1 -- Controlled Voltage Source7/LConn1
  C bus 5/RConn1 -- Controlled Current Source3/LConn1 -- Voltage bus 5/RConn2 -- Electrical Reference4/LConn1 -- Voltage output 5/RConn2 -- Solver Configuration1/RConn1 -- Controlled Voltage Source4/RConn2
  Voltage output 5/LConn1 -- Current output 5/LConn1 -- Controlled Voltage Source4/LConn1
  Controlled Voltage Source6/RConn2 -- Controlled Current Source2/LConn1 -- Voltage bus 8/RConn2 -- C bus 8/RConn1 -- Voltage output 8/RConn2 -- Electrical Reference7/LConn1
  Current output 12/LConn1 -- Voltage output 8/LConn1 -- Controlled Voltage Source6/LConn1
  R serie 8/RConn1 -- R serie 17/LConn1 -- R serie 15/LConn1 -- Current load 6/LConn1 -- Voltage bus 6/LConn1 -- C bus 6/LConn1 -- L serie 6/RConn1
  R serie 16/LConn1 -- R serie 17/RConn1 -- Current load 7/LConn1 -- R serie 9/RConn1 -- C bus 7/LConn1 -- L serie 7/RConn1 -- Voltage bus 7/LConn1
  PS-Simulink Converter35/LConn1 -- Voltage bus 8/RConn1
  R serie 14/LConn1 -- Current output 12/RConn2
  Controlled Current Source2/RConn2 -- Current load 8/RConn2
  Simulink-PS Converter13/RConn1 -- Controlled Voltage Source6/RConn1
  L serie 8/LConn1 -- R serie 14/RConn1
  Current load 8/RConn1 -- PS-Simulink Converter20/LConn1
  R serie 10/LConn1 -- Current output 8/RConn2
  R serie 7/LConn1 -- Current output 5/RConn2
  Simulink-PS Converter12/RConn1 -- Controlled Current Source2/RConn1
  Simulink-PS Converter6/RConn1 -- Controlled Current Source4/RConn1
  PS-Simulink Converter21/LConn1 -- Current output 8/RConn1
  L serie 5/LConn1 -- R serie 7/RConn1
  Simulink-PS Converter14/RConn1 -- Controlled Current Source3/RConn1
  Controlled Current Source4/RConn2 -- Current load 6/RConn2
  Current load 6/RConn1 -- PS-Simulink Converter24/LConn1
  PS-Simulink Converter33/LConn1 -- Current output 10/RConn1
  PS-Simulink Converter22/LConn1 -- Voltage output 6/RConn1
  Simulink-PS Converter15/RConn1 -- Controlled Voltage Source7/RConn1
  Current load 7/RConn1 -- PS-Simulink Converter26/LConn1
  Simulink-PS Converter5/RConn1 -- Controlled Current Source8/RConn1
  PS-Simulink Converter6/LConn1 -- Current output 5/RConn1
  L serie 7/LConn1 -- R serie 11/RConn1
  Simulink-PS Converter7/RConn1 -- Controlled Voltage Source5/RConn1
  PS-Simulink Converter31/LConn1 -- Voltage bus 5/RConn1
  Current output 10/RConn2 -- R serie 8/LConn1
  PS-Simulink Converter30/LConn1 -- Voltage output 7/RConn1
  PS-Simulink Converter29/LConn1 -- Current output 9/RConn1
  Simulink-PS Converter4/RConn1 -- Controlled Voltage Source4/RConn1
  Controlled Current Source3/RConn2 -- Current load 5/RConn2
  Current output 11/RConn2 -- R serie 9/LConn1
  R serie 11/LConn1 -- Current output 9/RConn2
  Controlled Current Source8/RConn2 -- Current load 7/RConn2
  PS-Simulink Converter23/LConn1 -- Voltage bus 6/RConn1
  PS-Simulink Converter27/LConn1 -- Current output 12/RConn1
  Current load 5/RConn1 -- PS-Simulink Converter32/LConn1
  PS-Simulink Converter19/LConn1 -- Voltage output 5/RConn1
  PS-Simulink Converter25/LConn1 -- Voltage bus 7/RConn1
  L serie 6/LConn1 -- R serie 10/RConn1
  Current output 11/RConn1 -- PS-Simulink Converter34/LConn1
  PS-Simulink Converter28/LConn1 -- Voltage output 8/RConn1
  Voltage output 10/RConn2 -- Controlled Current Source11/LConn1 -- Voltage bus 10/RConn2 -- C bus 10/RConn1 -- Electrical Reference9/LConn1 -- Controlled Voltage Source11/RConn2
  Controlled Voltage Source9/RConn2 -- Electrical Reference10/LConn1 -- Voltage output 11/RConn2 -- C bus 11/RConn1 -- Voltage bus 11/RConn2 -- Controlled Current Source12/LConn1
  Current output 15/LConn1 -- Controlled Voltage Source9/LConn1 -- Voltage output 11/LConn1
  Voltage bus 9/LConn1 -- Current output 16/LConn1 -- R serie 30/RConn1 -- R serie 27/RConn1 -- Current load 9/LConn1 -- Current output 17/LConn1 -- L serie 9/RConn1 -- C bus 9/LConn1
  Current output 14/LConn1 -- Voltage output 10/LConn1 -- Controlled Voltage Source11/LConn1
  C bus 9/RConn1 -- Controlled Current Source10/LConn1 -- Voltage bus 9/RConn2 -- Electrical Reference8/LConn1 -- Voltage output 9/RConn2 -- Solver Configuration2/RConn1 -- Controlled Voltage Source8/RConn2
  Voltage output 9/LConn1 -- Current output 13/LConn1 -- Controlled Voltage Source8/LConn1
  R serie 20/RConn1 -- Current load 10/LConn1 -- R serie 26/RConn1 -- Voltage bus 10/LConn1 -- C bus 10/LConn1 -- L serie 10/RConn1
  R serie 26/LConn1 -- Current load 11/LConn1 -- R serie 21/RConn1 -- C bus 11/LConn1 -- L serie 11/RConn1 -- Voltage bus 11/LConn1
  R serie 22/LConn1 -- Current output 14/RConn2
  Simulink-PS Converter16/RConn1 -- Controlled Voltage Source8/RConn1
  L serie 9/LConn1 -- R serie 19/RConn1
  PS-Simulink Converter39/LConn1 -- Current output 14/RConn1
  Current load 10/RConn1 -- PS-Simulink Converter42/LConn1
  Simulink-PS Converter22/RConn1 -- Controlled Current Source10/RConn1
  PS-Simulink Converter51/LConn1 -- Current output 16/RConn1
  R serie 19/LConn1 -- Current output 13/RConn2
  Current load 11/RConn1 -- PS-Simulink Converter44/LConn1
  Simulink-PS Converter23/RConn1 -- Controlled Voltage Source11/RConn1
  Simulink-PS Converter17/RConn1 -- Controlled Current Source12/RConn1
  PS-Simulink Converter36/LConn1 -- Current output 13/RConn1
  Simulink-PS Converter18/RConn1 -- Controlled Current Source11/RConn1
  Current output 16/RConn2 -- R serie 20/LConn1
  Simulink-PS Converter19/RConn1 -- Controlled Voltage Source9/RConn1
  PS-Simulink Converter47/LConn1 -- Current output 15/RConn1
  Controlled Current Source10/RConn2 -- Current load 9/RConn2
  Current output 17/RConn2 -- R serie 21/LConn1
  R serie 23/LConn1 -- Current output 15/RConn2
  Controlled Current Source12/RConn2 -- Current load 11/RConn2
  PS-Simulink Converter49/LConn1 -- Voltage bus 9/RConn1
  PS-Simulink Converter41/LConn1 -- Voltage bus 10/RConn1
  L serie 11/LConn1 -- R serie 23/RConn1
  Current load 9/RConn1 -- PS-Simulink Converter50/LConn1
  PS-Simulink Converter40/LConn1 -- Voltage output 10/RConn1
  PS-Simulink Converter37/LConn1 -- Voltage output 9/RConn1
  PS-Simulink Converter48/LConn1 -- Voltage output 11/RConn1
  Current output 17/RConn1 -- PS-Simulink Converter52/LConn1
  PS-Simulink Converter43/LConn1 -- Voltage bus 11/RConn1
  Controlled Current Source11/RConn2 -- Current load 10/RConn2
  L serie 10/LConn1 -- R serie 22/RConn1
  Controlled Current Source13/LConn1 -- Voltage output 12/RConn2 -- Controlled Voltage Source10/RConn2 -- Electrical Reference13/LConn1 -- C bus 12/RConn1 -- Voltage bus 12/RConn2
  L serie 14/RConn1 -- Voltage bus 14/LConn1 -- R serie 29/RConn1 -- Current load 14/LConn1 -- R serie 27/LConn1 -- Current output 21/LConn1 -- C bus 14/LConn1
  Voltage output 12/LConn1 -- Current output 19/LConn1 -- Controlled Voltage Source10/LConn1
  Solver Configuration3/RConn1 -- C bus 14/RConn1 -- Voltage bus 14/RConn2 -- Controlled Current Source9/LConn1 -- Voltage output 14/RConn2 -- Electrical Reference12/LConn1 -- Controlled Voltage Source12/RConn2
  Current output 18/LConn1 -- Voltage output 14/LConn1 -- Controlled Voltage Source12/LConn1
  C bus 12/LConn1 -- Current load 12/LConn1 -- R serie 25/RConn1 -- Voltage bus 12/LConn1 -- L serie 12/RConn1
  L serie 12/LConn1 -- R serie 28/RConn1
  Controlled Current Source13/RConn2 -- Current load 12/RConn2
  PS-Simulink Converter45/LConn1 -- Voltage output 14/RConn1
  Current load 14/RConn1 -- PS-Simulink Converter61/LConn1
  PS-Simulink Converter54/LConn1 -- Voltage bus 12/RConn1
  PS-Simulink Converter60/LConn1 -- Voltage bus 14/RConn1
  Controlled Current Source9/RConn2 -- Current load 14/RConn2
  Simulink-PS Converter24/RConn1 -- Controlled Current Source13/RConn1
  PS-Simulink Converter53/LConn1 -- Voltage output 12/RConn1
  PS-Simulink Converter62/LConn1 -- Current output 21/RConn1
  PS-Simulink Converter38/LConn1 -- Current output 18/RConn1
  Current load 12/RConn1 -- PS-Simulink Converter55/LConn1
  Current output 21/RConn2 -- R serie 25/LConn1
  L serie 14/LConn1 -- R serie 24/RConn1
  Simulink-PS Converter20/RConn1 -- Controlled Voltage Source12/RConn1
  R serie 24/LConn1 -- Current output 18/RConn2
  Simulink-PS Converter27/RConn1 -- Controlled Voltage Source10/RConn1
  R serie 28/LConn1 -- Current output 19/RConn2
  PS-Simulink Converter46/LConn1 -- Current output 19/RConn1
  Simulink-PS Converter26/RConn1 -- Controlled Current Source9/RConn1
